simulink model "bu_abslut125_rombina_32"  (R2021b)
(part 3 of 8)

  ROM6 : hdlBasic/ROM  depth=7874  initVector=[1,0,0,0,0,1,0,1,1,1,1,1,1,0,0,1,1,0,0,1,1,1,0,0,1,1,1,0,0,0,0,1,1,0,0,0,0,0,1,1,0,0,0,1,1,0,1,1,0,0,0,1,1,1,0,1,1,0,0,0,1,1,1,0,0,1,1,1,0,0,1,1,1,0,0,1,1,1,1,0,0,1,1,1,0,0,1,1,1,0,0,0,0,1,1,1,0,0,0,1,1,0,0,0,1,0,0,1,1,0,0,0,1,1,0,0,0,1,1,1,0,1,1,0,0,0,1,1,0,0,0,1,1,1,0,0,1,1,1,0,0,1,1,1,0,0,1,1,1,0,0,1,1,1,1,0,0,1,1,1,0,0,1,1,1,0,0,1,1,1,0,1,0,0,1,1,1,0,0,1,1,1,0,0,1,1,1,0,0,0,0,0,0,1,1,0,0,0,1,1,0,0,0,1,1,0,0,0,1,1,0,0,1,1,0,0,0,1,1,0,0,0,1,1,0,0,0,1,1,1,0,0,1,1,1,0,0,1,1,0,0,0,1,1,0,0,0,1,1,1,0,0,1,0,1,1,0,0,1,1,1,0,0,1,1,1,0,0,1,1,1,0,0,1,1,1,1,1,0,0,0,1,1,0,0,1,1,1,0,0,1,1,1,0,0,1,1,1,0,0,1,1,0,0,1,1,0,0,0,1,1,0,0,0,1,1,0,0,0,1,1,0,0,0,1,1,0,0,1,1,1,0,0,1,1,0,0,0,1,1,0,0,0,1,1,0,0,0,1,1,1,1,0,0,1,1,0,0,1,1,1,0,0,1,1,0,0,0,1,1,0,0,0,1,1,1,0,0,0,0,1,1,0,0,0,1,1,0,0,1,1,1,0,0,1,1,1,0,0,1,1,1,0,0,1,1,0,0,1,1,0,0,1,1,0,0,0,1,1,0,0,1,1,1,0,0,1,1,1,0,0,1,1,1,0,0,1,1,0,0,1,1,1,0,0,1,1,0,0,0,1,1,0,0,1,1,1,0,0,1,1,1,0,0,0,0,1,1,0,0,1,1,0,0,1,1,1,0,0,1,1,0,0,0,1,1,0,0,0,1,1,0,0,0,1,1,1,1,0,0,1,1,1,0,0,1,1,0,0,1,1,1,0,0,1,1,0,0,0,1,1,0,0,0,1,1,0,0,1,1,0,0,1,1,0,0,1,1,0,0,0,1,1,0,0,1,1,1,0,0,1,1,0,0,0,1,1,1,0,0,1,1,0,0,1,1,1,0,0,1,1,0,0,1,1,0,0,0,1,1,0,0,1,1,1,0,0,1,1,1,0,0,1,1,1,1,0,0,1,1,0,0,1,1,0,0,0,1,1,0,0,1,1,0,0,0,1,1,0,0,1,1,1,0,0,1,1,1,0,0,0,0,1,1,1,0,0,1,1,0,0,1,1,0,0,1,1,1,0,0,1,1,0,0,0,1,1,0,0,0,1,1,0,0,0,1,0,0,1,1,0,0,1,1,0,0,0,1,1,0,0,1,1,0,0,1,1,1,0,0,1,1,0,0,0,1,1,0,0,0,1,1,0,0,0,1,1,0,0,1,1,0,0,1,1,0,0,1,1,1,0,0,1,1,0,0,1,1,1,0,0,1,1,0,0,0,1,1,0,0,0,0,1,1,0,0,1,1,0,0,0,1,1,0,0,1,1,0,0,1,1,0,0,0,1,1,0,0,1,1,1,0,0,1,1,1,0,0,1,1,0,1,1,0,0,1,1,0,0,1,1,0,0,1,1,1,0,0,1,1,0,0,1,1,0,0,0,1,1,0,0,1,1,1,0,0,1,1,1,0,1,1,0,0,0,1,1,0,0,1,1,0,0,1,1,0,0,1,1,0,0,0,1,1,0,0,1,1,0,0,0,1,1,0,0,1,1,1,0,0,0,1,1,0,0,1,1,0,0,1,1,0,0,1,1,1,0,0,1,1,0,0,1,1,0,0,1,1,1,0,0,1,1,0,0,0,1,1,0,0,0,1,1,1,1,0,0,1,1,0,0,1,1,0,0,1,1,0,0,1,1,0,0,0,1,1,0,0,1,1,0,0,1,1,1,0,0,1,1,0,0,0,1,1,0,0,1,0,0,1,1,1,0,0,1,1,0,0,1,1,0,0,1,1,0,0,1,1,0,0,1,1,1,0,0,1,1,0,0,1,1,1,0,0,1,1,1,0,0,1,1,0,0,1,1,0,0,1,1,0,0,1,1,0,0,1,1,1,0,0,1,1,0,0,1,1,0,0,1,1,0,0,0,1,1,0,0,1,1,1,0,0,1,1,1,1,0,0,1,1,0,0,1,1,0,0,1,1,0,0,1,1,0,0,1,1,0,0,1,1,1,0,0,1,1,0,0,1,1,0,0,0,1,1,0,0,1,1,1,0,0,1,0,0,1,1,0,0,1,1,0,0,1,1,0,0,1,1,0,0,1,1,0,0,1,1,0,0,1,1,0,0,0,1,1,0,0,1,1,0,0,0,1,1,0,0,0,1,0,0,1,1,0,0,1,1,0,0,1,1,0,0,1,1,0,0,1,1,1,0,0,1,1,0,0,1,1,0,0,1,1,0,0,1,1,1,0,0,1,1,0,0,0,1,1,0,0,0,1,1,0,0,1,1,0,0,1,1,0,0,1,1,0,0,1,1,0,0,1,1,0,0,1,1,0,0,0,1,1,0,0,1,1,0,0,1,1,1,0,0,1,1,0,0,0,0,0,1,1,0,0,1,1,0,0,1,1,0,0,1,1,0,0,1,1,0,0,1,1,0,0,1,1,0,0,1,1,0,0,1,1,1,0,0,1,1,0,0,1,1,1,0,0,1,1,0,0,1,1,0,0,1,1,0,0,1,1,0,0,1,1,0,0,1,1,0,0,1,1,0,0,1,1,0,0,1,1,0,0,1,1,0,0,1,1,0,0,0,1,1,0,0,1,1,1,0,0,1,1,0,0,1,1,0,0,1,1,0,0,1,1,0,0,1,1,0,0,1,1,0,0,1,1,0,0,1,1,0,0,0,1,1,0,0,1,1,0,0,1,1,0,0,0,1,1,0,0,0,0,1,1,0,0,1,1,0,0,1,1,0,0,1,1,0,0,1,1,0,0,1,1,0,0,1,1,0,0,1,1,0,0,1,1,0,0,1,1,0,0,0,1,1,0,0,1,1,0,0,0,1,1,0,1,1,0,0,1,1,0,0,1,1,0,0,1,1,0,0,1,1,0,0,1,1,0,0,1,1,0,0,1,1,0,0,1,1,0,0,1,1,0,0,1,1,0,0,1,1,1,0,0,1,1,0,0,0,1,1,0,0,1,1,0,0,1,1,0,0,1,1,0,0,1,1,0,0,1,1,0,0,1,1,0,0,1,1,0,0,1,1,0,0,1,1,0,0,1,1,0,0,1,1,0,0,1,1,1,0,0,1,0,1,1,0,0,1,1,0,0,1,1,0,0,1,1,0,0,1,0,0,1,1,0,0,1,1,0,0,1,1,0,0,1,1,0,0,1,1,0,0,1,1,0,0,1,1,1,0,0,1,1,0,0,1,1,1,0,1,1,0,0,1,1,0,0,1,1,0,1,1,0,0,1,1,0,0,1,1,0,0,1,1,0,0,1,1,0,0,1,1,0,0,1,1,0,0,1,1,0,0,1,1,0,0,1,1,0,0,0,1,1,0,0,0,1,1,0,0,1,1,0,1,1,0,0,1,1,0,0,1,1,0,0,1,1,0,0,1,1,0,0,1,1,0,0,1,1,0,0,1,1,0,0,1,1,0,0,1,1,0,0,1,1,0,0,1,1,0,0,0,1,0,1,1,0,0,1,0,0,1,1,0,0,1,1,0,0,1,1,0,0,1,1,0,0,1,1,0,0,1,1,0,0,1,1,0,0,1,1,0,0,1,1,0,0,1,1,0,0,1,1,0,0,1,1,0,0,1,1,0,0,1,1,0,1,1,0,0,1,1,0,0,1,1,0,0,1,1,0,0,1,1,0,0,1,1,0,0,1,1,0,0,1,1,0,0,1,0,0,1,1,0,0,1,1,0,0,1,1,0,0,1,1,0,0,1,1,1,0,0,0,1,0,0,1,1,0,0,1,1,0,0,1,1,0,0,1,1,0,0,1,1,0,0,1,1,0,0,1,1,0,0,1,1,0,1,1,0,0,1,1,0,0,1,1,0,0,1,1,0,0,1,1,0,0,1,1,0,0,1,1,0,1,0,0,1,1,0,0,1,1,0,0,1,1,0,0,1,1,0,0,1,1,0,0,1,1,0,0,1,1,0,0,1,0,0,1,1,0,0,1,1,0,0,1,1,0,0,1,1,0,0,1,1,0,0,1,1,0,0,1,1,0,0,1,0,0,1,1,0,0,1,1,0,0,1,1,0,0,1,1,0,0,1,1,0,0,1,1,0,0,1,1,0,0,1,0,0,1,1,0,0,1,1,0,0,1,1,0 ...(+11750 chars)]  distributed_mem=Block RAM  rst=off  init_reg=0  en=off  latency=1  gui_display_data_type=Boolean  arith_type=Boolean  n_bits=2  bin_pt=0  preci_type=Double  exp_width=8  frac_width=24  optimize=Area  use_rpm=on  simulation_type=fast_sim  XmcBlockStatus=1  maskContainerNames=tabcontainer1  block_type=sprom  block_config=sysgen:SPROM_config
  ROM7 : hdlBasic/ROM  depth=7874  initVector=[0,1,1,1,0,1,0,1,0,0,1,0,0,1,0,0,0,1,0,1,1,0,1,0,1,1,0,1,1,0,0,1,0,1,1,0,0,0,1,0,1,1,0,1,0,0,1,0,1,1,0,1,0,0,1,1,0,1,1,0,1,0,0,1,0,1,0,0,1,0,1,0,0,1,0,1,1,0,0,1,0,1,1,0,1,0,1,1,0,1,0,1,0,1,1,0,1,0,0,1,0,1,1,0,1,0,0,1,0,1,0,0,1,0,1,1,0,1,0,0,0,1,0,1,1,0,1,0,1,1,0,1,0,0,1,0,1,0,0,1,0,1,0,0,1,0,1,0,0,1,0,1,1,1,0,1,0,1,0,0,1,0,1,0,0,1,0,1,1,0,1,0,1,0,1,1,0,1,0,1,1,0,1,0,1,1,0,1,0,0,1,1,0,1,0,1,0,0,1,0,1,0,0,1,0,1,0,0,1,0,1,0,1,0,1,1,0,1,0,1,0,0,1,0,1,1,0,1,0,0,1,0,1,1,0,1,0,1,0,1,1,0,1,0,1,1,0,1,0,0,1,0,1,0,1,0,1,0,1,1,0,1,0,1,0,0,1,0,1,0,0,1,0,1,1,0,1,0,1,1,0,1,0,1,0,1,1,0,1,0,1,1,0,1,0,1,1,0,1,0,1,0,1,0,1,0,1,1,0,1,0,1,0,0,1,0,1,0,0,1,0,1,0,0,1,0,1,0,1,1,0,1,0,1,0,1,1,0,1,0,1,0,0,1,0,1,1,0,1,0,0,0,1,0,1,0,1,0,1,0,0,1,0,1,0,1,1,0,1,0,1,1,0,1,0,0,1,0,1,0,1,0,1,1,0,1,0,1,0,1,1,0,1,0,1,0,0,1,0,1,0,0,1,0,1,1,0,0,1,0,1,0,1,0,1,0,0,1,0,1,0,1,1,0,1,0,1,0,0,1,0,1,1,0,1,0,1,0,1,0,1,1,0,1,0,1,0,1,0,0,1,0,1,0,1,1,0,1,0,1,1,0,1,0,0,0,1,0,1,0,1,0,1,0,1,1,0,1,0,1,0,1,0,0,1,0,1,0,0,1,0,1,0,0,1,0,1,0,1,0,1,0,0,1,0,1,0,1,0,1,0,0,1,0,1,0,1,1,0,1,0,1,1,0,1,0,1,1,1,0,1,0,1,0,1,0,1,0,1,1,0,1,0,1,0,1,0,0,1,0,1,0,1,1,0,1,0,0,1,0,1,0,1,0,1,0,0,1,0,1,0,1,0,1,0,1,1,0,1,0,1,0,1,1,0,1,0,1,0,0,1,0,1,1,0,0,1,0,1,0,1,0,1,0,1,0,0,1,0,1,0,1,0,1,0,0,1,0,1,0,1,1,0,1,0,1,1,0,1,0,1,0,1,0,0,1,0,1,0,1,0,1,0,1,0,1,1,0,1,0,1,0,1,0,0,1,0,1,0,0,1,0,1,0,0,1,1,0,1,0,1,0,1,0,1,0,0,1,0,1,0,1,0,1,0,1,0,0,1,0,1,0,1,1,0,1,0,1,0,0,1,0,1,1,0,1,0,1,0,1,0,1,0,1,0,1,0,1,0,0,1,0,1,0,1,0,1,0,0,1,0,1,0,1,1,0,1,0,1,1,0,0,1,0,1,0,1,0,1,0,0,1,0,1,0,1,0,1,0,1,0,1,1,0,1,0,1,0,1,0,0,1,0,1,0,0,1,0,1,1,0,1,0,1,0,1,0,1,0,1,0,1,0,1,0,0,1,0,1,0,1,0,1,0,1,0,0,1,0,1,0,1,1,0,1,0,1,1,0,1,1,0,1,0,0,1,0,1,0,1,0,1,0,1,0,1,0,1,0,1,0,0,1,0,1,0,1,0,1,0,0,1,0,1,0,1,1,0,1,0,0,1,0,1,0,1,0,1,0,1,0,1,0,1,1,0,1,0,1,0,1,0,1,0,1,0,1,1,0,1,0,1,0,1,0,0,1,0,1,0,0,1,0,1,0,1,0,1,0,1,0,1,0,1,0,1,0,1,0,1,0,1,0,0,1,0,1,0,1,0,1,0,1,0,0,1,0,1,0,1,1,0,1,0,1,1,0,1,0,1,1,0,1,0,1,0,1,0,1,0,1,0,1,0,1,0,1,0,1,0,1,0,0,1,0,1,0,1,0,1,0,0,1,0,1,0,0,1,0,1,0,1,0,1,0,1,0,1,0,1,0,1,0,1,0,1,0,0,1,0,1,0,1,0,1,0,1,0,1,0,1,1,0,1,0,1,0,1,0,0,1,0,1,1,0,0,1,0,1,0,1,0,1,0,1,0,1,0,1,0,1,0,1,0,1,0,1,0,1,0,0,1,0,1,0,1,0,1,0,1,0,0,1,0,1,0,1,1,0,1,0,0,1,0,1,0,1,0,1,0,1,0,1,0,1,0,1,0,1,0,1,0,1,0,1,0,1,0,1,0,1,0,0,1,0,1,0,1,0,1,0,0,1,0,1,0,0,1,1,0,1,0,1,0,1,0,1,0,1,0,1,0,1,0,1,0,1,1,0,1,0,1,0,1,0,1,0,1,0,1,0,1,0,1,0,0,1,0,1,0,1,0,0,1,0,1,1,0,1,0,1,0,1,0,1,0,1,0,1,0,1,0,1,0,1,0,1,0,1,0,1,0,1,0,1,1,0,1,0,1,0,1,0,1,0,1,0,0,1,0,1,0,1,1,0,1,0,1,0,1,0,1,0,1,0,1,0,1,0,1,0,1,0,1,0,1,0,1,0,1,0,1,0,1,0,1,0,1,0,1,0,0,1,0,1,0,1,0,1,0,0,1,0,1,0,1,0,1,0,1,0,1,0,1,0,1,0,1,0,1,0,1,0,1,0,1,0,1,0,1,0,1,0,1,0,1,0,1,0,1,0,1,0,1,0,1,0,0,1,0,1,0,1,1,0,1,0,1,0,1,0,1,0,1,0,1,0,1,0,1,0,1,0,1,0,1,0,1,0,1,0,1,0,1,0,1,0,1,0,0,1,0,1,0,1,0,1,0,1,0,1,0,0,1,0,1,0,0,0,1,0,1,0,1,0,1,0,1,0,1,0,1,0,1,0,1,0,1,0,1,0,1,0,1,0,1,0,1,0,1,0,1,0,1,0,1,0,1,0,0,1,0,1,0,1,0,1,0,0,1,0,0,1,0,1,0,1,0,1,0,1,0,1,0,1,0,1,0,1,0,1,0,1,0,1,0,1,0,1,0,1,0,1,0,1,0,1,0,1,0,1,0,1,0,1,0,1,0,0,1,0,1,0,1,1,0,1,0,1,0,1,0,1,0,1,0,1,0,1,0,1,0,1,0,1,0,1,0,1,0,1,0,1,0,1,0,1,0,1,0,1,0,1,0,1,0,1,0,1,0,1,0,1,0,1,0,0,1,0,1,0,1,0,1,0,1,0,1,0,1,0,1,0,1,0,1,0,1,1,0,1,0,1,0,1,0,1,0,1,0,1,0,1,0,1,0,1,0,1,0,1,0,1,0,1,0,0,1,0,1,0,1,0,1,0,0,0,1,0,1,0,1,0,1,0,1,0,1,1,0,1,0,1,0,1,0,1,0,1,0,1,0,1,0,1,0,1,0,1,0,1,0,1,0,1,0,1,0,1,0,1,0,1,0,1,0,1,0,0,1,0,1,0,0,1,0,1,0,1,0,1,1,0,1,0,1,0,1,0,1,0,1,0,1,0,1,0,1,0,1,0,1,0,1,0,1,0,1,0,1,0,1,0,1,0,1,0,1,0,1,0,1,0,1,0,1,0,1,0,0,1,0,1,0,1,0,0,1,0,1,0,1,0,1,0,1,0,1,0,1,0,1,0,1,0,1,0,1,0,1,0,1,0,1,0,1,0,1,0,1,0,1,0,1,0,1,0,1,0,1,0,1,0,1,0,1,0,1,0,1,0,1,0,0,1,0,1,0,1,0,1,0,1,0,1,0,1,0,1,0,1,0,1,0,1,0,1,0,1,0,1,0,1,0,1,0,1,1,0,1,0,1,0,1,0,1,0,1,0,1,0,1,0,1,0,1,0,0,1,0,0,1,1,0,1,0,1,0,1,0,1,0,1,0,1,0,1,0,1,0,1,0,1,0,1,0,1,0,1,0,1,0,1,0,0,1,0,1,0,1,0,1,0,1,0,1,0,1,0,1,0,1,0,1,0,1,0,1,0,1,0,0,0,1,0,1,0,1,0,1,0,1,0,1,0,1,0,1,0,1,0,1,0,1,0,1,0,1,0,1,0,1,0,0,1,0,1,0,1,0,1,0,1,0,1,0,1,0,1,0,1,0,1,0,1,0,1,0,1,0,1,0,1,0,0,1,0,1,0,1,0,1,0,1,0,1,0,1,0,1,0,1,0,1,0,1,0,1,0,1,0,1,0,1,0,0,1,0,1,0,1,0,1,0,1,0,1,0,1 ...(+11750 chars)]  distributed_mem=Block RAM  rst=off  init_reg=0  en=off  latency=1  gui_display_data_type=Boolean  arith_type=Boolean  n_bits=2  bin_pt=0  preci_type=Double  exp_width=8  frac_width=24  optimize=Area  use_rpm=on  simulation_type=fast_sim  XmcBlockStatus=1  maskContainerNames=tabcontainer1  block_type=sprom  block_config=sysgen:SPROM_config
  ROM8 : hdlBasic/ROM  depth=7874  initVector=[1,1,0,0,0,1,0,1,1,0,1,1,0,0,1,1,0,0,1,1,0,0,0,1,1,0,0,1,1,1,0,0,1,1,0,0,1,0,0,1,1,0,0,1,1,0,0,1,1,0,0,1,1,0,0,1,1,1,0,0,1,1,0,0,1,1,1,0,0,1,1,1,0,0,1,1,0,0,0,0,1,1,0,0,0,1,1,0,0,1,1,1,1,1,0,0,1,1,0,0,1,1,0,0,1,1,0,0,1,1,1,0,0,1,1,0,0,1,1,0,0,0,1,1,0,0,0,1,1,0,0,1,1,0,0,1,1,1,0,0,0,1,1,0,0,0,1,1,0,0,1,1,0,0,0,0,1,1,1,0,0,1,1,1,0,0,1,1,0,0,1,0,1,1,1,0,0,1,1,1,0,0,1,1,1,0,0,1,1,0,1,0,0,0,1,1,1,0,0,0,1,1,0,0,1,1,1,0,1,1,0,0,1,1,1,0,0,0,1,1,1,0,0,1,1,0,0,1,1,0,0,1,1,0,0,0,0,1,1,1,0,0,1,1,1,0,0,1,1,0,0,1,1,0,0,0,1,1,1,0,0,0,1,1,1,0,0,0,1,1,0,0,1,1,0,0,1,1,1,0,0,0,0,1,1,1,0,0,0,1,1,0,0,0,1,1,0,0,1,1,0,0,0,0,1,1,1,0,0,0,0,1,1,0,0,0,1,1,0,0,0,1,1,0,0,1,1,1,1,0,0,0,0,1,1,1,0,0,0,1,1,1,0,0,1,1,0,0,0,1,0,0,0,0,0,0,1,1,1,1,0,0,0,1,1,1,0,0,0,1,1,0,0,1,1,0,0,1,0,1,1,1,1,0,0,0,0,1,1,1,0,0,0,0,1,1,0,0,0,1,1,0,0,1,1,0,1,0,0,0,0,1,1,1,1,1,0,0,0,1,1,1,0,0,0,1,1,1,0,0,1,1,0,0,1,1,1,1,1,1,1,0,0,0,0,1,1,1,1,0,0,0,1,1,1,0,0,1,1,1,0,0,1,1,0,0,0,0,0,0,0,1,1,1,1,0,0,0,0,1,1,1,1,0,0,1,1,1,0,0,0,1,1,0,0,1,1,1,1,1,1,1,0,0,0,0,0,1,1,1,1,0,0,0,1,1,1,0,0,0,1,1,0,0,0,1,1,0,0,0,0,0,0,0,1,1,1,1,1,0,0,0,0,1,1,1,1,0,0,0,1,1,1,0,0,1,1,0,0,1,1,1,1,1,1,1,0,0,0,0,0,0,1,1,1,1,0,0,0,0,1,1,1,0,0,0,1,1,1,0,0,1,1,0,0,0,0,0,0,0,1,1,1,1,1,1,0,0,0,0,0,1,1,1,1,0,0,0,1,1,1,0,0,0,1,1,0,0,1,1,1,1,1,1,0,0,0,0,0,0,0,1,1,1,1,1,0,0,0,0,1,1,1,1,0,0,0,1,1,0,0,0,1,1,0,0,0,0,1,1,1,1,1,1,1,1,0,0,0,0,0,0,1,1,1,1,1,0,0,0,1,1,1,0,0,0,1,1,1,0,0,1,1,0,0,0,0,0,0,0,0,0,0,1,1,1,1,1,1,0,0,0,0,0,1,1,1,1,0,0,0,1,1,1,0,0,1,1,1,0,0,1,1,1,1,1,1,1,1,1,0,0,0,0,0,0,0,1,1,1,1,1,0,0,0,0,1,1,1,1,0,0,0,1,1,0,0,1,1,0,0,0,0,0,0,0,0,1,1,1,1,1,1,1,1,0,0,0,0,0,0,1,1,1,1,1,0,0,0,1,1,1,0,0,0,1,1,0,0,1,1,1,1,1,0,0,0,0,0,0,0,0,0,0,1,1,1,1,1,1,1,0,0,0,0,0,1,1,1,1,0,0,0,1,1,1,0,0,1,1,0,1,1,1,1,1,1,1,1,1,1,1,1,1,0,0,0,0,0,0,0,0,1,1,1,1,1,0,0,0,0,1,1,1,1,0,0,0,1,1,0,0,1,0,0,0,0,0,0,0,0,0,0,1,1,1,1,1,1,1,1,1,1,0,0,0,0,0,0,1,1,1,1,1,0,0,0,1,1,1,0,0,0,1,1,0,1,1,1,1,0,0,0,0,0,0,0,0,0,0,0,0,0,0,0,1,1,1,1,1,1,1,0,0,0,0,0,1,1,1,1,0,0,0,1,1,0,0,0,1,1,1,1,1,1,1,1,1,1,1,1,1,1,1,1,1,1,0,0,0,0,0,0,0,0,0,1,1,1,1,1,0,0,0,0,0,1,1,1,0,0,1,1,0,0,0,0,0,0,0,0,0,0,0,0,0,0,1,1,1,1,1,1,1,1,1,1,1,1,1,0,0,0,0,0,0,0,1,1,1,1,0,0,0,1,1,1,0,0,1,1,0,0,0,0,0,0,0,0,0,0,0,0,0,0,0,0,0,0,0,0,0,0,0,1,1,1,1,1,1,1,1,0,0,0,0,0,1,1,1,1,0,0,0,1,1,0,0,1,1,1,1,1,1,1,1,1,1,1,1,1,1,1,1,1,1,1,0,0,0,0,0,0,0,0,0,0,0,0,1,1,1,1,1,1,0,0,0,0,1,1,1,0,0,1,1,1,1,1,1,1,1,1,1,1,1,1,1,1,1,1,1,1,1,1,1,1,1,1,1,1,1,1,1,1,0,0,0,0,0,0,0,0,1,1,1,1,0,0,0,1,1,1,0,0,0,0,0,0,0,0,0,0,0,0,0,0,0,0,0,0,0,0,0,0,0,0,0,0,0,0,1,1,1,1,1,1,1,1,1,1,0,0,0,0,0,0,1,1,1,0,0,0,1,1,0,0,0,0,0,0,0,0,0,0,0,0,0,0,0,0,0,0,0,0,0,0,0,0,0,0,0,0,0,0,0,0,0,0,0,0,1,1,1,1,1,1,0,0,0,0,1,1,0,0,1,1,1,1,1,1,1,1,1,1,1,1,1,1,1,1,1,1,1,1,1,1,1,1,1,1,1,1,1,1,1,1,1,1,0,0,0,0,0,0,0,0,0,1,1,1,1,0,0,0,1,1,0,1,1,1,1,1,1,1,1,1,1,1,1,1,1,1,1,1,1,1,1,1,1,1,1,1,1,1,1,1,1,1,1,1,1,1,1,1,1,1,1,1,0,0,0,0,0,0,1,1,1,0,0,1,1,1,1,1,1,1,1,1,1,0,0,0,0,0,0,0,0,0,0,0,0,0,0,0,0,0,0,0,0,0,0,0,0,0,0,0,0,0,0,0,1,1,1,1,1,1,1,0,0,0,0,1,1,0,1,1,0,0,0,0,0,0,0,0,0,0,0,0,0,0,0,0,0,0,0,0,0,0,0,0,0,0,0,0,0,0,0,0,0,0,0,0,0,0,0,0,0,0,0,0,0,1,1,1,1,0,0,0,1,0,0,0,0,0,0,0,0,0,0,0,0,0,0,0,0,0,0,1,1,1,1,1,1,1,1,1,1,1,1,1,1,1,1,1,1,1,1,1,1,1,1,1,1,1,1,0,0,0,0,0,0,1,1,1,0,0,0,0,0,0,0,0,0,0,0,0,0,1,1,1,1,1,1,1,1,1,1,1,1,1,1,1,1,1,1,1,1,1,1,1,1,1,1,1,1,1,1,1,1,1,1,1,1,1,1,1,1,0,0,0,1,1,0,0,0,0,0,0,0,0,1,1,1,1,1,1,1,1,1,1,1,1,1,1,1,1,1,1,1,0,0,0,0,0,0,0,0,0,0,0,0,0,0,0,0,0,0,0,0,0,0,0,0,0,1,1,1,1,0,0,0,0,0,0,0,1,1,1,1,1,1,1,1,1,1,1,1,1,1,1,1,1,0,0,0,0,0,0,0,0,0,0,0,0,0,0,0,0,0,0,0,0,0,0,0,0,0,0,0,0,0,0,0,0,0,0,0,1,1,0,0,0,1,1,1,1,1,1,1,1,1,1,1,1,1,1,1,1,0,0,0,0,0,0,0,0,0,0,0,0,0,0,0,0,0,0,1,1,1,1,1,1,1,1,1,1,1,1,1,1,1,1,1,1,1,1,0,0,0,0,0,1,1,1,1,1,1,1,1,1,1,1,1,1,1,1,0,0,0,0,0,0,0,0,0,0,0,0,0,0,0,0,0,1,1,1,1,1,1,1,1,1,1,1,1,1,1,1,1,1,1,1,1,1,1,1,1,1,1,1,0,1,1,1,1,1,1,1,1,1,1,1,1,1,1,1,0,0,0,0,0,0,0,0,0,0,0,0,0,0,0,0,1,1,1,1,1,1,1,1,1,1,1,1,1,1,1,1,0,0,0,0,0,0,0,0,0,0,0,0,0,0,0,1,1,1,1,1,1,1,1,1,1,1,1,1,1,1,0,0,0,0,0,0,0,0,0,0,0,0,0,0,0,0,1,1,1,1,1,1,1,1,1,1,1,1,1,1 ...(+11750 chars)]  distributed_mem=Block RAM  rst=off  init_reg=0  en=off  latency=1  gui_display_data_type=Boolean  arith_type=Boolean  n_bits=2  bin_pt=0  preci_type=Double  exp_width=8  frac_width=24  optimize=Area  use_rpm=on  simulation_type=fast_sim  XmcBlockStatus=1  maskContainerNames=tabcontainer1  block_type=sprom  block_config=sysgen:SPROM_config
  ROM9 : hdlBasic/ROM  depth=7874  initVector=[0,1,0,0,1,0,1,0,1,0,0,1,0,1,0,1,0,1,0,1,0,0,1,0,1,0,1,1,0,1,0,1,0,1,0,1,1,0,1,0,1,0,1,0,1,0,1,0,1,0,1,0,1,0,1,0,0,1,0,1,0,1,0,1,0,1,1,0,1,0,0,1,0,1,0,1,0,1,0,1,0,1,0,1,1,0,1,0,1,0,1,0,1,1,0,1,0,1,0,1,0,1,0,1,0,1,0,1,0,0,1,0,1,0,1,0,1,0,1,0,1,1,0,1,0,1,1,0,1,0,1,0,1,0,1,0,0,1,0,0,1,0,1,0,0,1,0,1,0,1,0,1,0,0,0,1,0,1,1,0,1,0,1,1,0,1,0,1,0,1,0,1,0,1,1,0,1,0,0,1,0,1,0,1,1,0,1,0,1,0,1,0,0,1,0,0,1,0,1,1,0,1,0,1,0,1,1,0,0,1,1,1,0,1,1,0,1,1,0,1,1,0,1,0,1,0,1,0,1,0,1,0,1,0,0,1,1,0,1,1,0,1,0,0,1,0,1,0,1,0,1,0,1,0,1,1,0,0,1,0,0,1,0,0,1,0,1,1,0,1,0,1,0,1,0,1,0,0,1,0,0,1,1,0,1,1,0,1,1,0,1,0,1,1,0,1,0,1,0,1,0,0,1,1,0,0,1,0,0,1,1,0,1,0,0,1,0,1,0,0,1,0,1,0,1,0,0,1,1,0,0,1,1,0,0,1,0,0,1,0,0,1,0,1,0,1,0,0,1,0,0,0,0,0,1,1,0,0,1,1,0,1,1,0,1,1,0,1,1,0,1,0,1,0,1,0,1,0,1,0,0,1,1,0,0,1,1,0,0,1,0,0,1,1,0,1,0,0,1,0,1,0,1,0,1,0,1,0,0,1,1,0,0,0,1,1,0,1,1,0,0,1,0,0,1,0,1,1,0,1,0,1,0,1,0,0,0,0,1,1,1,0,0,1,1,0,0,1,1,0,1,1,0,1,1,0,1,0,0,1,0,1,0,1,0,0,0,0,1,1,1,0,0,1,1,0,0,1,1,0,0,1,1,0,1,0,0,1,0,1,1,0,1,0,1,0,0,0,0,1,1,1,0,0,1,1,1,0,0,1,1,0,1,1,0,0,1,0,0,1,0,1,0,1,1,0,1,1,0,0,0,1,1,1,0,0,1,1,1,0,0,1,1,0,0,1,1,0,1,1,0,1,1,0,1,0,1,0,1,0,1,0,0,1,1,1,0,0,0,1,1,1,0,0,1,1,0,0,1,1,0,0,1,0,0,1,0,0,1,0,1,0,1,0,1,0,1,1,1,1,0,0,0,1,1,1,0,0,1,1,1,0,0,1,1,0,1,1,0,0,1,0,1,1,0,1,0,1,0,1,1,1,1,1,0,0,0,0,1,1,1,0,0,1,1,1,0,0,1,1,0,0,1,1,0,1,1,0,1,0,0,1,0,1,0,1,1,1,0,0,0,0,0,1,1,1,0,0,0,1,1,1,0,0,1,1,1,0,0,1,0,0,1,0,0,1,0,1,1,0,1,0,1,0,0,0,0,0,0,1,1,1,1,0,0,0,1,1,1,0,0,0,1,1,0,0,1,1,0,0,1,0,0,1,0,1,0,0,1,0,1,0,0,0,0,1,1,1,1,1,0,0,0,1,1,1,1,0,0,0,1,1,0,0,1,1,0,0,1,1,0,1,1,0,1,0,1,0,1,0,1,1,1,1,1,1,1,0,0,0,0,1,1,1,1,0,0,0,1,1,1,0,0,0,1,1,0,0,1,0,0,1,0,0,1,0,1,0,1,0,1,1,1,1,0,0,0,0,0,0,1,1,1,1,0,0,0,0,1,1,1,0,0,0,1,1,0,0,1,1,0,0,1,0,1,1,0,1,0,1,0,0,0,0,0,0,0,0,1,1,1,1,1,1,0,0,0,0,1,1,1,1,0,0,0,1,1,0,0,1,1,0,0,1,1,0,1,1,0,1,0,1,0,0,1,1,1,1,1,1,1,1,1,0,0,0,0,0,0,1,1,1,1,0,0,0,0,1,1,0,0,0,1,1,0,0,1,0,0,1,0,0,1,0,1,0,1,1,1,1,0,0,0,0,0,0,0,0,0,1,1,1,1,1,1,0,0,0,0,1,1,1,0,0,0,1,1,0,0,1,1,0,0,1,0,1,0,0,1,0,0,0,0,0,0,0,0,0,1,1,1,1,1,1,1,1,1,0,0,0,0,0,1,1,1,1,0,0,0,1,1,0,0,0,1,1,0,1,1,0,1,0,1,0,1,1,1,1,1,1,1,1,1,1,1,1,1,0,0,0,0,0,0,0,0,1,1,1,1,1,0,0,0,0,1,1,1,0,0,1,1,0,0,1,0,0,1,0,1,0,1,0,0,0,0,0,0,0,0,0,0,0,0,0,0,0,1,1,1,1,1,1,1,1,0,0,0,0,0,1,1,1,0,0,0,1,1,0,0,1,1,0,1,1,0,1,0,1,1,1,1,1,1,1,1,1,1,1,1,1,1,1,1,1,1,1,1,0,0,0,0,0,0,0,1,1,1,1,1,0,0,0,1,1,1,0,0,1,1,0,1,1,0,1,0,1,0,0,0,0,0,0,0,0,0,0,0,0,0,0,0,0,0,0,0,0,0,0,0,1,1,1,1,1,1,0,0,0,0,0,1,1,1,0,0,1,1,0,0,1,0,0,1,0,1,1,1,1,1,1,1,1,1,1,1,1,1,1,1,1,1,1,1,1,1,1,1,1,1,1,1,0,0,0,0,0,0,1,1,1,1,0,0,0,1,1,1,0,1,1,0,1,1,0,1,0,0,0,0,0,0,0,0,0,0,0,0,0,0,0,0,0,0,0,0,0,0,0,0,0,0,0,0,0,0,1,1,1,1,1,1,0,0,0,1,1,1,0,0,1,1,0,1,0,1,0,1,1,1,1,1,1,1,1,1,1,1,1,1,1,1,1,1,1,1,1,1,1,1,1,1,1,1,1,1,1,1,1,1,0,0,0,0,0,1,1,1,1,0,0,1,1,0,0,1,0,1,0,1,1,1,1,1,0,0,0,0,0,0,0,0,0,0,0,0,0,0,0,0,0,0,0,0,0,0,0,0,0,0,0,0,0,0,0,1,1,1,1,1,0,0,0,1,1,1,0,1,1,0,1,0,0,0,0,0,0,0,0,0,0,1,1,1,1,1,1,1,1,1,1,1,1,1,1,1,1,1,1,1,1,1,1,1,1,1,1,1,1,1,1,1,0,0,0,0,1,1,1,0,0,1,1,0,1,0,0,0,1,1,1,1,1,1,1,1,1,1,1,1,0,0,0,0,0,0,0,0,0,0,0,0,0,0,0,0,0,0,0,0,0,0,0,0,0,0,0,0,0,1,1,1,1,0,0,1,1,0,0,1,0,1,1,1,1,1,1,1,0,0,0,0,0,0,0,0,0,0,0,1,1,1,1,1,1,1,1,1,1,1,1,1,1,1,1,1,1,1,1,1,1,1,1,1,1,1,1,0,0,0,0,1,1,0,1,1,0,1,1,0,0,0,0,0,0,0,0,0,0,1,1,1,1,1,1,1,1,1,1,1,0,0,0,0,0,0,0,0,0,0,0,0,0,0,0,0,0,0,0,0,0,0,0,0,0,0,1,1,1,0,0,1,0,1,0,0,0,0,0,0,0,0,1,1,1,1,1,1,1,1,1,0,0,0,0,0,0,0,0,0,0,1,1,1,1,1,1,1,1,1,1,1,1,1,1,1,1,1,1,1,1,1,1,1,1,1,0,0,0,1,0,1,0,0,0,0,0,1,1,1,1,1,1,1,1,0,0,0,0,0,0,0,0,0,1,1,1,1,1,1,1,1,1,1,0,0,0,0,0,0,0,0,0,0,0,0,0,0,0,0,0,0,0,0,0,0,0,1,1,0,1,0,0,0,1,1,1,1,1,1,1,1,0,0,0,0,0,0,0,0,1,1,1,1,1,1,1,1,1,0,0,0,0,0,0,0,0,0,1,1,1,1,1,1,1,1,1,1,1,1,1,1,1,1,1,1,1,1,0,0,1,0,0,1,1,1,1,1,1,1,0,0,0,0,0,0,0,0,1,1,1,1,1,1,1,1,0,0,0,0,0,0,0,0,0,1,1,1,1,1,1,1,1,0,0,0,0,0,0,0,0,0,0,0,0,0,0,0,0,0,0,1,0,1,1,1,1,1,1,1,1,0,0,0,0,0,0,0,1,1,1,1,1,1,1,1,0,0,0,0,0,0,0,0,1,1,1,1,1,1,1,1,0,0,0,0,0,0,0,0,1,1,1,1,1,1,1,1,1,1,1,1,1,1,0,1,1,1,1,1,1,1,0,0,0,0,0,0,0,0,1,1,1,1,1,1,1,1,0,0,0,0,0,0,0,0,1,1,1,1,1,1,1,0,0,0,0,0,0,0 ...(+11750 chars)]  distributed_mem=Block RAM  rst=off  init_reg=0  en=off  latency=1  gui_display_data_type=Boolean  arith_type=Boolean  n_bits=2  bin_pt=0  preci_type=Double  exp_width=8  frac_width=24  optimize=Area  use_rpm=on  simulation_type=fast_sim  XmcBlockStatus=1  maskContainerNames=tabcontainer1  block_type=sprom  block_config=sysgen:SPROM_config
  Relational : hdlBasic/Relational  mode=a<b  op_type=Bool  en=off  latency=1  XmcBlockStatus=1  maskContainerNames=tabcontainer1  block_type=relational  block_config=sysgen:Relational_config
  Relational{1..92,95..118,120..122,124..208,210,238..239,250,253,258..262,264..273,275..284,286..295,297..302} (250 alike) : hdlBasic/Relational  mode=a>=b  op_type=Bool  en=off  latency=1  XmcBlockStatus=1  maskContainerNames=tabcontainer1  block_type=relational  block_config=sysgen:Relational_config
  Scaling : hdlBasic/Scale  scale_factor=-31  XmcBlockStatus=1  maskContainerNames=group1  block_type=scale  block_config=sysgen:Scale_config
  Slice : hdlBasic/Slice  nbits=7  boolean_output=off  mode=Lower Bit Location + Width  bit1=-1  base1=MSB of Input  bit0=0  base0=LSB of Input  XmcBlockStatus=1  maskContainerNames=group1  block_type=slice  block_config=sysgen:Slice_config
  Slice1 : hdlBasic/Slice  nbits=7  boolean_output=off  mode=Lower Bit Location + Width  bit1=-1  base1=MSB of Input  bit0=0  base0=LSB of Input  XmcBlockStatus=1  maskContainerNames=group1  block_type=slice  block_config=sysgen:Slice_config
  Slice2 : hdlBasic/Slice  nbits=21  boolean_output=off  mode=Two Bit Locations  bit1=-1  base1=MSB of Input  bit0=1  base0=LSB of Input  XmcBlockStatus=1  maskContainerNames=group1  block_type=slice  block_config=sysgen:Slice_config
  Slice3 : hdlBasic/Slice  nbits=21  boolean_output=off  mode=Two Bit Locations  bit1=-4  base1=MSB of Input  bit0=0  base0=LSB of Input  XmcBlockStatus=1  maskContainerNames=group1  block_type=slice  block_config=sysgen:Slice_config
  logi_b0 : hdlBasic/Constant  const=-1.0000000000000000000000000000000000000000000000000000000  gui_display_data_type=Fixed-point  arith_type=Signed (2's comp)  n_bits=32  bin_pt=30  preci_type=Double  exp_width=8  frac_width=24  explicit_period=on  period=1  XmcBlockStatus=1  maskContainerNames=tabcontainer1  block_type=constant  block_config=sysgen:Constant_config
  logi_b1 : hdlBasic/Constant  const=-0.9838709677419354981964261241955682635307312011718750000  gui_display_data_type=Fixed-point  arith_type=Signed (2's comp)  n_bits=32  bin_pt=30  preci_type=Double  exp_width=8  frac_width=24  explicit_period=on  period=1  XmcBlockStatus=1  maskContainerNames=tabcontainer1  block_type=constant  block_config=sysgen:Constant_config
  logi_b10 : hdlBasic/Constant  const=-0.8387096774193547599196563169243745505809783935546875000  gui_display_data_type=Fixed-point  arith_type=Signed (2's comp)  n_bits=32  bin_pt=30  preci_type=Double  exp_width=8  frac_width=24  explicit_period=on  period=1  XmcBlockStatus=1  maskContainerNames=tabcontainer1  block_type=constant  block_config=sysgen:Constant_config
  logi_b100 : hdlBasic/Constant  const=0.6129032258064516236473195931466761976480484008789062500  gui_display_data_type=Fixed-point  arith_type=Signed (2's comp)  n_bits=32  bin_pt=30  preci_type=Double  exp_width=8  frac_width=24  explicit_period=on  period=1  XmcBlockStatus=1  maskContainerNames=tabcontainer1  block_type=constant  block_config=sysgen:Constant_config
  logi_b101 : hdlBasic/Constant  const=0.6290322580645161254508934689511079341173171997070312500  gui_display_data_type=Fixed-point  arith_type=Signed (2's comp)  n_bits=32  bin_pt=30  preci_type=Double  exp_width=8  frac_width=24  explicit_period=on  period=1  XmcBlockStatus=1  maskContainerNames=tabcontainer1  block_type=constant  block_config=sysgen:Constant_config
  logi_b102 : hdlBasic/Constant  const=0.6451612903225806272544673447555396705865859985351562500  gui_display_data_type=Fixed-point  arith_type=Signed (2's comp)  n_bits=32  bin_pt=30  preci_type=Double  exp_width=8  frac_width=24  explicit_period=on  period=1  XmcBlockStatus=1  maskContainerNames=tabcontainer1  block_type=constant  block_config=sysgen:Constant_config
  logi_b103 : hdlBasic/Constant  const=0.6612903225806451290580412205599714070558547973632812500  gui_display_data_type=Fixed-point  arith_type=Signed (2's comp)  n_bits=32  bin_pt=30  preci_type=Double  exp_width=8  frac_width=24  explicit_period=on  period=1  XmcBlockStatus=1  maskContainerNames=tabcontainer1  block_type=constant  block_config=sysgen:Constant_config
  logi_b104 : hdlBasic/Constant  const=0.6774193548387096308616150963644031435251235961914062500  gui_display_data_type=Fixed-point  arith_type=Signed (2's comp)  n_bits=32  bin_pt=30  preci_type=Double  exp_width=8  frac_width=24  explicit_period=on  period=1  XmcBlockStatus=1  maskContainerNames=tabcontainer1  block_type=constant  block_config=sysgen:Constant_config
  logi_b105 : hdlBasic/Constant  const=0.6935483870967741326651889721688348799943923950195312500  gui_display_data_type=Fixed-point  arith_type=Signed (2's comp)  n_bits=32  bin_pt=30  preci_type=Double  exp_width=8  frac_width=24  explicit_period=on  period=1  XmcBlockStatus=1  maskContainerNames=tabcontainer1  block_type=constant  block_config=sysgen:Constant_config
  logi_b106 : hdlBasic/Constant  const=0.7096774193548387454910653104889206588268280029296875000  gui_display_data_type=Fixed-point  arith_type=Signed (2's comp)  n_bits=32  bin_pt=30  preci_type=Double  exp_width=8  frac_width=24  explicit_period=on  period=1  XmcBlockStatus=1  maskContainerNames=tabcontainer1  block_type=constant  block_config=sysgen:Constant_config
  logi_b107 : hdlBasic/Constant  const=0.7258064516129032472946391862933523952960968017578125000  gui_display_data_type=Fixed-point  arith_type=Signed (2's comp)  n_bits=32  bin_pt=30  preci_type=Double  exp_width=8  frac_width=24  explicit_period=on  period=1  XmcBlockStatus=1  maskContainerNames=tabcontainer1  block_type=constant  block_config=sysgen:Constant_config
  logi_b108 : hdlBasic/Constant  const=0.7419354838709677490982130620977841317653656005859375000  gui_display_data_type=Fixed-point  arith_type=Signed (2's comp)  n_bits=32  bin_pt=30  preci_type=Double  exp_width=8  frac_width=24  explicit_period=on  period=1  XmcBlockStatus=1  maskContainerNames=tabcontainer1  block_type=constant  block_config=sysgen:Constant_config
  logi_b109 : hdlBasic/Constant  const=0.7580645161290322509017869379022158682346343994140625000  gui_display_data_type=Fixed-point  arith_type=Signed (2's comp)  n_bits=32  bin_pt=30  preci_type=Double  exp_width=8  frac_width=24  explicit_period=on  period=1  XmcBlockStatus=1  maskContainerNames=tabcontainer1  block_type=constant  block_config=sysgen:Constant_config
  logi_b11 : hdlBasic/Constant  const=-0.8225806451612902581160824411199428141117095947265625000  gui_display_data_type=Fixed-point  arith_type=Signed (2's comp)  n_bits=32  bin_pt=30  preci_type=Double  exp_width=8  frac_width=24  explicit_period=on  period=1  XmcBlockStatus=1  maskContainerNames=tabcontainer1  block_type=constant  block_config=sysgen:Constant_config
  logi_b110 : hdlBasic/Constant  const=0.7741935483870967527053608137066476047039031982421875000  gui_display_data_type=Fixed-point  arith_type=Signed (2's comp)  n_bits=32  bin_pt=30  preci_type=Double  exp_width=8  frac_width=24  explicit_period=on  period=1  XmcBlockStatus=1  maskContainerNames=tabcontainer1  block_type=constant  block_config=sysgen:Constant_config
  logi_b111 : hdlBasic/Constant  const=0.7903225806451612545089346895110793411731719970703125000  gui_display_data_type=Fixed-point  arith_type=Signed (2's comp)  n_bits=32  bin_pt=30  preci_type=Double  exp_width=8  frac_width=24  explicit_period=on  period=1  XmcBlockStatus=1  maskContainerNames=tabcontainer1  block_type=constant  block_config=sysgen:Constant_config
  logi_b112 : hdlBasic/Constant  const=0.8064516129032257563125085653155110776424407958984375000  gui_display_data_type=Fixed-point  arith_type=Signed (2's comp)  n_bits=32  bin_pt=30  preci_type=Double  exp_width=8  frac_width=24  explicit_period=on  period=1  XmcBlockStatus=1  maskContainerNames=tabcontainer1  block_type=constant  block_config=sysgen:Constant_config
  logi_b113 : hdlBasic/Constant  const=0.8225806451612902581160824411199428141117095947265625000  gui_display_data_type=Fixed-point  arith_type=Signed (2's comp)  n_bits=32  bin_pt=30  preci_type=Double  exp_width=8  frac_width=24  explicit_period=on  period=1  XmcBlockStatus=1  maskContainerNames=tabcontainer1  block_type=constant  block_config=sysgen:Constant_config
  logi_b114 : hdlBasic/Constant  const=0.8387096774193547599196563169243745505809783935546875000  gui_display_data_type=Fixed-point  arith_type=Signed (2's comp)  n_bits=32  bin_pt=30  preci_type=Double  exp_width=8  frac_width=24  explicit_period=on  period=1  XmcBlockStatus=1  maskContainerNames=tabcontainer1  block_type=constant  block_config=sysgen:Constant_config
  logi_b115 : hdlBasic/Constant  const=0.8548387096774193727455326552444603294134140014648437500  gui_display_data_type=Fixed-point  arith_type=Signed (2's comp)  n_bits=32  bin_pt=30  preci_type=Double  exp_width=8  frac_width=24  explicit_period=on  period=1  XmcBlockStatus=1  maskContainerNames=tabcontainer1  block_type=constant  block_config=sysgen:Constant_config
  logi_b116 : hdlBasic/Constant  const=0.8709677419354838745491065310488920658826828002929687500  gui_display_data_type=Fixed-point  arith_type=Signed (2's comp)  n_bits=32  bin_pt=30  preci_type=Double  exp_width=8  frac_width=24  explicit_period=on  period=1  XmcBlockStatus=1  maskContainerNames=tabcontainer1  block_type=constant  block_config=sysgen:Constant_config
  logi_b117 : hdlBasic/Constant  const=0.8870967741935483763526804068533238023519515991210937500  gui_display_data_type=Fixed-point  arith_type=Signed (2's comp)  n_bits=32  bin_pt=30  preci_type=Double  exp_width=8  frac_width=24  explicit_period=on  period=1  XmcBlockStatus=1  maskContainerNames=tabcontainer1  block_type=constant  block_config=sysgen:Constant_config
  logi_b118 : hdlBasic/Constant  const=0.9032258064516128781562542826577555388212203979492187500  gui_display_data_type=Fixed-point  arith_type=Signed (2's comp)  n_bits=32  bin_pt=30  preci_type=Double  exp_width=8  frac_width=24  explicit_period=on  period=1  XmcBlockStatus=1  maskContainerNames=tabcontainer1  block_type=constant  block_config=sysgen:Constant_config
  logi_b119 : hdlBasic/Constant  const=0.9193548387096773799598281584621872752904891967773437500  gui_display_data_type=Fixed-point  arith_type=Signed (2's comp)  n_bits=32  bin_pt=30  preci_type=Double  exp_width=8  frac_width=24  explicit_period=on  period=1  XmcBlockStatus=1  maskContainerNames=tabcontainer1  block_type=constant  block_config=sysgen:Constant_config
  logi_b12 : hdlBasic/Constant  const=-0.8064516129032257563125085653155110776424407958984375000  gui_display_data_type=Fixed-point  arith_type=Signed (2's comp)  n_bits=32  bin_pt=30  preci_type=Double  exp_width=8  frac_width=24  explicit_period=on  period=1  XmcBlockStatus=1  maskContainerNames=tabcontainer1  block_type=constant  block_config=sysgen:Constant_config
  logi_b120 : hdlBasic/Constant  const=0.9354838709677418817634020342666190117597579956054687500  gui_display_data_type=Fixed-point  arith_type=Signed (2's comp)  n_bits=32  bin_pt=30  preci_type=Double  exp_width=8  frac_width=24  explicit_period=on  period=1  XmcBlockStatus=1  maskContainerNames=tabcontainer1  block_type=constant  block_config=sysgen:Constant_config
  logi_b121 : hdlBasic/Constant  const=0.9516129032258063835669759100710507482290267944335937500  gui_display_data_type=Fixed-point  arith_type=Signed (2's comp)  n_bits=32  bin_pt=30  preci_type=Double  exp_width=8  frac_width=24  explicit_period=on  period=1  XmcBlockStatus=1  maskContainerNames=tabcontainer1  block_type=constant  block_config=sysgen:Constant_config
  logi_b122 : hdlBasic/Constant  const=0.9677419354838709963928522483911365270614624023437500000  gui_display_data_type=Fixed-point  arith_type=Signed (2's comp)  n_bits=32  bin_pt=30  preci_type=Double  exp_width=8  frac_width=24  explicit_period=on  period=1  XmcBlockStatus=1  maskContainerNames=tabcontainer1  block_type=constant  block_config=sysgen:Constant_config
  logi_b123 : hdlBasic/Constant  const=0.9838709677419354981964261241955682635307312011718750000  gui_display_data_type=Fixed-point  arith_type=Signed (2's comp)  n_bits=32  bin_pt=30  preci_type=Double  exp_width=8  frac_width=24  explicit_period=on  period=1  XmcBlockStatus=1  maskContainerNames=tabcontainer1  block_type=constant  block_config=sysgen:Constant_config
  logi_b124 : hdlBasic/Constant  const=1.0000000000000000000000000000000000000000000000000000000  gui_display_data_type=Fixed-point  arith_type=Signed (2's comp)  n_bits=32  bin_pt=30  preci_type=Double  exp_width=8  frac_width=24  explicit_period=on  period=1  XmcBlockStatus=1  maskContainerNames=tabcontainer1  block_type=constant  block_config=sysgen:Constant_config
  logi_b13 : hdlBasic/Constant  const=-0.7903225806451612545089346895110793411731719970703125000  gui_display_data_type=Fixed-point  arith_type=Signed (2's comp)  n_bits=32  bin_pt=30  preci_type=Double  exp_width=8  frac_width=24  explicit_period=on  period=1  XmcBlockStatus=1  maskContainerNames=tabcontainer1  block_type=constant  block_config=sysgen:Constant_config
  logi_b14 : hdlBasic/Constant  const=-0.7741935483870967527053608137066476047039031982421875000  gui_display_data_type=Fixed-point  arith_type=Signed (2's comp)  n_bits=32  bin_pt=30  preci_type=Double  exp_width=8  frac_width=24  explicit_period=on  period=1  XmcBlockStatus=1  maskContainerNames=tabcontainer1  block_type=constant  block_config=sysgen:Constant_config
  logi_b15 : hdlBasic/Constant  const=-0.7580645161290322509017869379022158682346343994140625000  gui_display_data_type=Fixed-point  arith_type=Signed (2's comp)  n_bits=32  bin_pt=30  preci_type=Double  exp_width=8  frac_width=24  explicit_period=on  period=1  XmcBlockStatus=1  maskContainerNames=tabcontainer1  block_type=constant  block_config=sysgen:Constant_config
  logi_b16 : hdlBasic/Constant  const=-0.7419354838709677490982130620977841317653656005859375000  gui_display_data_type=Fixed-point  arith_type=Signed (2's comp)  n_bits=32  bin_pt=30  preci_type=Double  exp_width=8  frac_width=24  explicit_period=on  period=1  XmcBlockStatus=1  maskContainerNames=tabcontainer1  block_type=constant  block_config=sysgen:Constant_config
  logi_b17 : hdlBasic/Constant  const=-0.7258064516129032472946391862933523952960968017578125000  gui_display_data_type=Fixed-point  arith_type=Signed (2's comp)  n_bits=32  bin_pt=30  preci_type=Double  exp_width=8  frac_width=24  explicit_period=on  period=1  XmcBlockStatus=1  maskContainerNames=tabcontainer1  block_type=constant  block_config=sysgen:Constant_config
  logi_b18 : hdlBasic/Constant  const=-0.7096774193548387454910653104889206588268280029296875000  gui_display_data_type=Fixed-point  arith_type=Signed (2's comp)  n_bits=32  bin_pt=30  preci_type=Double  exp_width=8  frac_width=24  explicit_period=on  period=1  XmcBlockStatus=1  maskContainerNames=tabcontainer1  block_type=constant  block_config=sysgen:Constant_config
  logi_b19 : hdlBasic/Constant  const=-0.6935483870967741326651889721688348799943923950195312500  gui_display_data_type=Fixed-point  arith_type=Signed (2's comp)  n_bits=32  bin_pt=30  preci_type=Double  exp_width=8  frac_width=24  explicit_period=on  period=1  XmcBlockStatus=1  maskContainerNames=tabcontainer1  block_type=constant  block_config=sysgen:Constant_config
  logi_b2 : hdlBasic/Constant  const=-0.9677419354838709963928522483911365270614624023437500000  gui_display_data_type=Fixed-point  arith_type=Signed (2's comp)  n_bits=32  bin_pt=30  preci_type=Double  exp_width=8  frac_width=24  explicit_period=on  period=1  XmcBlockStatus=1  maskContainerNames=tabcontainer1  block_type=constant  block_config=sysgen:Constant_config
  logi_b20 : hdlBasic/Constant  const=-0.6774193548387096308616150963644031435251235961914062500  gui_display_data_type=Fixed-point  arith_type=Signed (2's comp)  n_bits=32  bin_pt=30  preci_type=Double  exp_width=8  frac_width=24  explicit_period=on  period=1  XmcBlockStatus=1  maskContainerNames=tabcontainer1  block_type=constant  block_config=sysgen:Constant_config
  logi_b21 : hdlBasic/Constant  const=-0.6612903225806451290580412205599714070558547973632812500  gui_display_data_type=Fixed-point  arith_type=Signed (2's comp)  n_bits=32  bin_pt=30  preci_type=Double  exp_width=8  frac_width=24  explicit_period=on  period=1  XmcBlockStatus=1  maskContainerNames=tabcontainer1  block_type=constant  block_config=sysgen:Constant_config
  logi_b22 : hdlBasic/Constant  const=-0.6451612903225806272544673447555396705865859985351562500  gui_display_data_type=Fixed-point  arith_type=Signed (2's comp)  n_bits=32  bin_pt=30  preci_type=Double  exp_width=8  frac_width=24  explicit_period=on  period=1  XmcBlockStatus=1  maskContainerNames=tabcontainer1  block_type=constant  block_config=sysgen:Constant_config
  logi_b23 : hdlBasic/Constant  const=-0.6290322580645161254508934689511079341173171997070312500  gui_display_data_type=Fixed-point  arith_type=Signed (2's comp)  n_bits=32  bin_pt=30  preci_type=Double  exp_width=8  frac_width=24  explicit_period=on  period=1  XmcBlockStatus=1  maskContainerNames=tabcontainer1  block_type=constant  block_config=sysgen:Constant_config
  logi_b24 : hdlBasic/Constant  const=-0.6129032258064516236473195931466761976480484008789062500  gui_display_data_type=Fixed-point  arith_type=Signed (2's comp)  n_bits=32  bin_pt=30  preci_type=Double  exp_width=8  frac_width=24  explicit_period=on  period=1  XmcBlockStatus=1  maskContainerNames=tabcontainer1  block_type=constant  block_config=sysgen:Constant_config
  logi_b25 : hdlBasic/Constant  const=-0.5967741935483871218437457173422444611787796020507812500  gui_display_data_type=Fixed-point  arith_type=Signed (2's comp)  n_bits=32  bin_pt=30  preci_type=Double  exp_width=8  frac_width=24  explicit_period=on  period=1  XmcBlockStatus=1  maskContainerNames=tabcontainer1  block_type=constant  block_config=sysgen:Constant_config
  logi_b26 : hdlBasic/Constant  const=-0.5806451612903225090178693790221586823463439941406250000  gui_display_data_type=Fixed-point  arith_type=Signed (2's comp)  n_bits=32  bin_pt=30  preci_type=Double  exp_width=8  frac_width=24  explicit_period=on  period=1  XmcBlockStatus=1  maskContainerNames=tabcontainer1  block_type=constant  block_config=sysgen:Constant_config
  logi_b27 : hdlBasic/Constant  const=-0.5645161290322580072142955032177269458770751953125000000  gui_display_data_type=Fixed-point  arith_type=Signed (2's comp)  n_bits=32  bin_pt=30  preci_type=Double  exp_width=8  frac_width=24  explicit_period=on  period=1  XmcBlockStatus=1  maskContainerNames=tabcontainer1  block_type=constant  block_config=sysgen:Constant_config
  logi_b28 : hdlBasic/Constant  const=-0.5483870967741935054107216274132952094078063964843750000  gui_display_data_type=Fixed-point  arith_type=Signed (2's comp)  n_bits=32  bin_pt=30  preci_type=Double  exp_width=8  frac_width=24  explicit_period=on  period=1  XmcBlockStatus=1  maskContainerNames=tabcontainer1  block_type=constant  block_config=sysgen:Constant_config
  logi_b29 : hdlBasic/Constant  const=-0.5322580645161290036071477516088634729385375976562500000  gui_display_data_type=Fixed-point  arith_type=Signed (2's comp)  n_bits=32  bin_pt=30  preci_type=Double  exp_width=8  frac_width=24  explicit_period=on  period=1  XmcBlockStatus=1  maskContainerNames=tabcontainer1  block_type=constant  block_config=sysgen:Constant_config
  logi_b3 : hdlBasic/Constant  const=-0.9516129032258063835669759100710507482290267944335937500  gui_display_data_type=Fixed-point  arith_type=Signed (2's comp)  n_bits=32  bin_pt=30  preci_type=Double  exp_width=8  frac_width=24  explicit_period=on  period=1  XmcBlockStatus=1  maskContainerNames=tabcontainer1  block_type=constant  block_config=sysgen:Constant_config
  logi_b30 : hdlBasic/Constant  const=-0.5161290322580645018035738758044317364692687988281250000  gui_display_data_type=Fixed-point  arith_type=Signed (2's comp)  n_bits=32  bin_pt=30  preci_type=Double  exp_width=8  frac_width=24  explicit_period=on  period=1  XmcBlockStatus=1  maskContainerNames=tabcontainer1  block_type=constant  block_config=sysgen:Constant_config
  logi_b31 : hdlBasic/Constant  const=-0.5000000000000000000000000000000000000000000000000000000  gui_display_data_type=Fixed-point  arith_type=Signed (2's comp)  n_bits=32  bin_pt=30  preci_type=Double  exp_width=8  frac_width=24  explicit_period=on  period=1  XmcBlockStatus=1  maskContainerNames=tabcontainer1  block_type=constant  block_config=sysgen:Constant_config
  logi_b32 : hdlBasic/Constant  const=-0.4838709677419354981964261241955682635307312011718750000  gui_display_data_type=Fixed-point  arith_type=Signed (2's comp)  n_bits=32  bin_pt=30  preci_type=Double  exp_width=8  frac_width=24  explicit_period=on  period=1  XmcBlockStatus=1  maskContainerNames=tabcontainer1  block_type=constant  block_config=sysgen:Constant_config
  logi_b33 : hdlBasic/Constant  const=-0.4677419354838709408817010171333095058798789978027343750  gui_display_data_type=Fixed-point  arith_type=Signed (2's comp)  n_bits=32  bin_pt=30  preci_type=Double  exp_width=8  frac_width=24  explicit_period=on  period=1  XmcBlockStatus=1  maskContainerNames=tabcontainer1  block_type=constant  block_config=sysgen:Constant_config
  logi_b34 : hdlBasic/Constant  const=-0.4516129032258064390781271413288777694106101989746093750  gui_display_data_type=Fixed-point  arith_type=Signed (2's comp)  n_bits=32  bin_pt=30  preci_type=Double  exp_width=8  frac_width=24  explicit_period=on  period=1  XmcBlockStatus=1  maskContainerNames=tabcontainer1  block_type=constant  block_config=sysgen:Constant_config
  logi_b35 : hdlBasic/Constant  const=-0.4354838709677419372745532655244460329413414001464843750  gui_display_data_type=Fixed-point  arith_type=Signed (2's comp)  n_bits=32  bin_pt=30  preci_type=Double  exp_width=8  frac_width=24  explicit_period=on  period=1  XmcBlockStatus=1  maskContainerNames=tabcontainer1  block_type=constant  block_config=sysgen:Constant_config
  logi_b36 : hdlBasic/Constant  const=-0.4193548387096773799598281584621872752904891967773437500  gui_display_data_type=Fixed-point  arith_type=Signed (2's comp)  n_bits=32  bin_pt=30  preci_type=Double  exp_width=8  frac_width=24  explicit_period=on  period=1  XmcBlockStatus=1  maskContainerNames=tabcontainer1  block_type=constant  block_config=sysgen:Constant_config
  logi_b37 : hdlBasic/Constant  const=-0.4032258064516128781562542826577555388212203979492187500  gui_display_data_type=Fixed-point  arith_type=Signed (2's comp)  n_bits=32  bin_pt=30  preci_type=Double  exp_width=8  frac_width=24  explicit_period=on  period=1  XmcBlockStatus=1  maskContainerNames=tabcontainer1  block_type=constant  block_config=sysgen:Constant_config
  logi_b38 : hdlBasic/Constant  const=-0.3870967741935483763526804068533238023519515991210937500  gui_display_data_type=Fixed-point  arith_type=Signed (2's comp)  n_bits=32  bin_pt=30  preci_type=Double  exp_width=8  frac_width=24  explicit_period=on  period=1  XmcBlockStatus=1  maskContainerNames=tabcontainer1  block_type=constant  block_config=sysgen:Constant_config
  logi_b39 : hdlBasic/Constant  const=-0.3709677419354838745491065310488920658826828002929687500  gui_display_data_type=Fixed-point  arith_type=Signed (2's comp)  n_bits=32  bin_pt=30  preci_type=Double  exp_width=8  frac_width=24  explicit_period=on  period=1  XmcBlockStatus=1  maskContainerNames=tabcontainer1  block_type=constant  block_config=sysgen:Constant_config
  logi_b4 : hdlBasic/Constant  const=-0.9354838709677418817634020342666190117597579956054687500  gui_display_data_type=Fixed-point  arith_type=Signed (2's comp)  n_bits=32  bin_pt=30  preci_type=Double  exp_width=8  frac_width=24  explicit_period=on  period=1  XmcBlockStatus=1  maskContainerNames=tabcontainer1  block_type=constant  block_config=sysgen:Constant_config
  logi_b40 : hdlBasic/Constant  const=-0.3548387096774193727455326552444603294134140014648437500  gui_display_data_type=Fixed-point  arith_type=Signed (2's comp)  n_bits=32  bin_pt=30  preci_type=Double  exp_width=8  frac_width=24  explicit_period=on  period=1  XmcBlockStatus=1  maskContainerNames=tabcontainer1  block_type=constant  block_config=sysgen:Constant_config
  logi_b41 : hdlBasic/Constant  const=-0.3387096774193548154308075481822015717625617980957031250  gui_display_data_type=Fixed-point  arith_type=Signed (2's comp)  n_bits=32  bin_pt=30  preci_type=Double  exp_width=8  frac_width=24  explicit_period=on  period=1  XmcBlockStatus=1  maskContainerNames=tabcontainer1  block_type=constant  block_config=sysgen:Constant_config
  logi_b42 : hdlBasic/Constant  const=-0.3225806451612903136272336723777698352932929992675781250  gui_display_data_type=Fixed-point  arith_type=Signed (2's comp)  n_bits=32  bin_pt=30  preci_type=Double  exp_width=8  frac_width=24  explicit_period=on  period=1  XmcBlockStatus=1  maskContainerNames=tabcontainer1  block_type=constant  block_config=sysgen:Constant_config
  logi_b43 : hdlBasic/Constant  const=-0.3064516129032258118236597965733380988240242004394531250  gui_display_data_type=Fixed-point  arith_type=Signed (2's comp)  n_bits=32  bin_pt=30  preci_type=Double  exp_width=8  frac_width=24  explicit_period=on  period=1  XmcBlockStatus=1  maskContainerNames=tabcontainer1  block_type=constant  block_config=sysgen:Constant_config
  logi_b44 : hdlBasic/Constant  const=-0.2903225806451612545089346895110793411731719970703125000  gui_display_data_type=Fixed-point  arith_type=Signed (2's comp)  n_bits=32  bin_pt=30  preci_type=Double  exp_width=8  frac_width=24  explicit_period=on  period=1  XmcBlockStatus=1  maskContainerNames=tabcontainer1  block_type=constant  block_config=sysgen:Constant_config
  logi_b45 : hdlBasic/Constant  const=-0.2741935483870967527053608137066476047039031982421875000  gui_display_data_type=Fixed-point  arith_type=Signed (2's comp)  n_bits=32  bin_pt=30  preci_type=Double  exp_width=8  frac_width=24  explicit_period=on  period=1  XmcBlockStatus=1  maskContainerNames=tabcontainer1  block_type=constant  block_config=sysgen:Constant_config
  logi_b46 : hdlBasic/Constant  const=-0.2580645161290322509017869379022158682346343994140625000  gui_display_data_type=Fixed-point  arith_type=Signed (2's comp)  n_bits=32  bin_pt=30  preci_type=Double  exp_width=8  frac_width=24  explicit_period=on  period=1  XmcBlockStatus=1  maskContainerNames=tabcontainer1  block_type=constant  block_config=sysgen:Constant_config
  logi_b47 : hdlBasic/Constant  const=-0.2419354838709677490982130620977841317653656005859375000  gui_display_data_type=Fixed-point  arith_type=Signed (2's comp)  n_bits=32  bin_pt=30  preci_type=Double  exp_width=8  frac_width=24  explicit_period=on  period=1  XmcBlockStatus=1  maskContainerNames=tabcontainer1  block_type=constant  block_config=sysgen:Constant_config
  logi_b48 : hdlBasic/Constant  const=-0.2258064516129032195390635706644388847053050994873046875  gui_display_data_type=Fixed-point  arith_type=Signed (2's comp)  n_bits=32  bin_pt=30  preci_type=Double  exp_width=8  frac_width=24  explicit_period=on  period=1  XmcBlockStatus=1  maskContainerNames=tabcontainer1  block_type=constant  block_config=sysgen:Constant_config
  logi_b49 : hdlBasic/Constant  const=-0.2096774193548386899799140792310936376452445983886718750  gui_display_data_type=Fixed-point  arith_type=Signed (2's comp)  n_bits=32  bin_pt=30  preci_type=Double  exp_width=8  frac_width=24  explicit_period=on  period=1  XmcBlockStatus=1  maskContainerNames=tabcontainer1  block_type=constant  block_config=sysgen:Constant_config
  logi_b5 : hdlBasic/Constant  const=-0.9193548387096773799598281584621872752904891967773437500  gui_display_data_type=Fixed-point  arith_type=Signed (2's comp)  n_bits=32  bin_pt=30  preci_type=Double  exp_width=8  frac_width=24  explicit_period=on  period=1  XmcBlockStatus=1  maskContainerNames=tabcontainer1  block_type=constant  block_config=sysgen:Constant_config
  logi_b50 : hdlBasic/Constant  const=-0.1935483870967741881763402034266619011759757995605468750  gui_display_data_type=Fixed-point  arith_type=Signed (2's comp)  n_bits=32  bin_pt=30  preci_type=Double  exp_width=8  frac_width=24  explicit_period=on  period=1  XmcBlockStatus=1  maskContainerNames=tabcontainer1  block_type=constant  block_config=sysgen:Constant_config
  logi_b51 : hdlBasic/Constant  const=-0.1774193548387096863727663276222301647067070007324218750  gui_display_data_type=Fixed-point  arith_type=Signed (2's comp)  n_bits=32  bin_pt=30  preci_type=Double  exp_width=8  frac_width=24  explicit_period=on  period=1  XmcBlockStatus=1  maskContainerNames=tabcontainer1  block_type=constant  block_config=sysgen:Constant_config
  logi_b52 : hdlBasic/Constant  const=-0.1612903225806451568136168361888849176466464996337890625  gui_display_data_type=Fixed-point  arith_type=Signed (2's comp)  n_bits=32  bin_pt=30  preci_type=Double  exp_width=8  frac_width=24  explicit_period=on  period=1  XmcBlockStatus=1  maskContainerNames=tabcontainer1  block_type=constant  block_config=sysgen:Constant_config
  logi_b53 : hdlBasic/Constant  const=-0.1451612903225806272544673447555396705865859985351562500  gui_display_data_type=Fixed-point  arith_type=Signed (2's comp)  n_bits=32  bin_pt=30  preci_type=Double  exp_width=8  frac_width=24  explicit_period=on  period=1  XmcBlockStatus=1  maskContainerNames=tabcontainer1  block_type=constant  block_config=sysgen:Constant_config
  logi_b54 : hdlBasic/Constant  const=-0.1290322580645161254508934689511079341173171997070312500  gui_display_data_type=Fixed-point  arith_type=Signed (2's comp)  n_bits=32  bin_pt=30  preci_type=Double  exp_width=8  frac_width=24  explicit_period=on  period=1  XmcBlockStatus=1  maskContainerNames=tabcontainer1  block_type=constant  block_config=sysgen:Constant_config
  logi_b55 : hdlBasic/Constant  const=-0.1129032258064516097695317853322194423526525497436523438  gui_display_data_type=Fixed-point  arith_type=Signed (2's comp)  n_bits=32  bin_pt=30  preci_type=Double  exp_width=8  frac_width=24  explicit_period=on  period=1  XmcBlockStatus=1  maskContainerNames=tabcontainer1  block_type=constant  block_config=sysgen:Constant_config
  logi_b56 : hdlBasic/Constant  const=-0.0967741935483870940881701017133309505879878997802734375  gui_display_data_type=Fixed-point  arith_type=Signed (2's comp)  n_bits=32  bin_pt=30  preci_type=Double  exp_width=8  frac_width=24  explicit_period=on  period=1  XmcBlockStatus=1  maskContainerNames=tabcontainer1  block_type=constant  block_config=sysgen:Constant_config
  logi_b57 : hdlBasic/Constant  const=-0.0806451612903225784068084180944424588233232498168945312  gui_display_data_type=Fixed-point  arith_type=Signed (2's comp)  n_bits=32  bin_pt=30  preci_type=Double  exp_width=8  frac_width=24  explicit_period=on  period=1  XmcBlockStatus=1  maskContainerNames=tabcontainer1  block_type=constant  block_config=sysgen:Constant_config
  logi_b58 : hdlBasic/Constant  const=-0.0645161290322580627254467344755539670586585998535156250  gui_display_data_type=Fixed-point  arith_type=Signed (2's comp)  n_bits=32  bin_pt=30  preci_type=Double  exp_width=8  frac_width=24  explicit_period=on  period=1  XmcBlockStatus=1  maskContainerNames=tabcontainer1  block_type=constant  block_config=sysgen:Constant_config
  logi_b59 : hdlBasic/Constant  const=-0.0483870967741935470440850508566654752939939498901367188  gui_display_data_type=Fixed-point  arith_type=Signed (2's comp)  n_bits=32  bin_pt=30  preci_type=Double  exp_width=8  frac_width=24  explicit_period=on  period=1  XmcBlockStatus=1  maskContainerNames=tabcontainer1  block_type=constant  block_config=sysgen:Constant_config
  logi_b6 : hdlBasic/Constant  const=-0.9032258064516128781562542826577555388212203979492187500  gui_display_data_type=Fixed-point  arith_type=Signed (2's comp)  n_bits=32  bin_pt=30  preci_type=Double  exp_width=8  frac_width=24  explicit_period=on  period=1  XmcBlockStatus=1  maskContainerNames=tabcontainer1  block_type=constant  block_config=sysgen:Constant_config
  logi_b60 : hdlBasic/Constant  const=-0.0322580645161290313627233672377769835293292999267578125  gui_display_data_type=Fixed-point  arith_type=Signed (2's comp)  n_bits=32  bin_pt=30  preci_type=Double  exp_width=8  frac_width=24  explicit_period=on  period=1  XmcBlockStatus=1  maskContainerNames=tabcontainer1  block_type=constant  block_config=sysgen:Constant_config
  logi_b61 : hdlBasic/Constant  const=-0.0161290322580645156813616836188884917646646499633789062  gui_display_data_type=Fixed-point  arith_type=Signed (2's comp)  n_bits=32  bin_pt=30  preci_type=Double  exp_width=8  frac_width=24  explicit_period=on  period=1  XmcBlockStatus=1  maskContainerNames=tabcontainer1  block_type=constant  block_config=sysgen:Constant_config
  logi_b62 : hdlBasic/Constant  const=0.0000000000000000000000000000000000000000000000000000000  gui_display_data_type=Fixed-point  arith_type=Signed (2's comp)  n_bits=32  bin_pt=30  preci_type=Double  exp_width=8  frac_width=24  explicit_period=on  period=1  XmcBlockStatus=1  maskContainerNames=tabcontainer1  block_type=constant  block_config=sysgen:Constant_config
  logi_b63 : hdlBasic/Constant  const=0.0161290322580645156813616836188884917646646499633789062  gui_display_data_type=Fixed-point  arith_type=Signed (2's comp)  n_bits=32  bin_pt=30  preci_type=Double  exp_width=8  frac_width=24  explicit_period=on  period=1  XmcBlockStatus=1  maskContainerNames=tabcontainer1  block_type=constant  block_config=sysgen:Constant_config
  logi_b64 : hdlBasic/Constant  const=0.0322580645161290313627233672377769835293292999267578125  gui_display_data_type=Fixed-point  arith_type=Signed (2's comp)  n_bits=32  bin_pt=30  preci_type=Double  exp_width=8  frac_width=24  explicit_period=on  period=1  XmcBlockStatus=1  maskContainerNames=tabcontainer1  block_type=constant  block_config=sysgen:Constant_config
  logi_b65 : hdlBasic/Constant  const=0.0483870967741935470440850508566654752939939498901367188  gui_display_data_type=Fixed-point  arith_type=Signed (2's comp)  n_bits=32  bin_pt=30  preci_type=Double  exp_width=8  frac_width=24  explicit_period=on  period=1  XmcBlockStatus=1  maskContainerNames=tabcontainer1  block_type=constant  block_config=sysgen:Constant_config
  logi_b66 : hdlBasic/Constant  const=0.0645161290322580627254467344755539670586585998535156250  gui_display_data_type=Fixed-point  arith_type=Signed (2's comp)  n_bits=32  bin_pt=30  preci_type=Double  exp_width=8  frac_width=24  explicit_period=on  period=1  XmcBlockStatus=1  maskContainerNames=tabcontainer1  block_type=constant  block_config=sysgen:Constant_config
  logi_b67 : hdlBasic/Constant  const=0.0806451612903225784068084180944424588233232498168945312  gui_display_data_type=Fixed-point  arith_type=Signed (2's comp)  n_bits=32  bin_pt=30  preci_type=Double  exp_width=8  frac_width=24  explicit_period=on  period=1  XmcBlockStatus=1  maskContainerNames=tabcontainer1  block_type=constant  block_config=sysgen:Constant_config
  logi_b68 : hdlBasic/Constant  const=0.0967741935483870940881701017133309505879878997802734375  gui_display_data_type=Fixed-point  arith_type=Signed (2's comp)  n_bits=32  bin_pt=30  preci_type=Double  exp_width=8  frac_width=24  explicit_period=on  period=1  XmcBlockStatus=1  maskContainerNames=tabcontainer1  block_type=constant  block_config=sysgen:Constant_config
  logi_b69 : hdlBasic/Constant  const=0.1129032258064516097695317853322194423526525497436523438  gui_display_data_type=Fixed-point  arith_type=Signed (2's comp)  n_bits=32  bin_pt=30  preci_type=Double  exp_width=8  frac_width=24  explicit_period=on  period=1  XmcBlockStatus=1  maskContainerNames=tabcontainer1  block_type=constant  block_config=sysgen:Constant_config
  logi_b7 : hdlBasic/Constant  const=-0.8870967741935483763526804068533238023519515991210937500  gui_display_data_type=Fixed-point  arith_type=Signed (2's comp)  n_bits=32  bin_pt=30  preci_type=Double  exp_width=8  frac_width=24  explicit_period=on  period=1  XmcBlockStatus=1  maskContainerNames=tabcontainer1  block_type=constant  block_config=sysgen:Constant_config
  logi_b70 : hdlBasic/Constant  const=0.1290322580645161254508934689511079341173171997070312500  gui_display_data_type=Fixed-point  arith_type=Signed (2's comp)  n_bits=32  bin_pt=30  preci_type=Double  exp_width=8  frac_width=24  explicit_period=on  period=1  XmcBlockStatus=1  maskContainerNames=tabcontainer1  block_type=constant  block_config=sysgen:Constant_config
  logi_b71 : hdlBasic/Constant  const=0.1451612903225806272544673447555396705865859985351562500  gui_display_data_type=Fixed-point  arith_type=Signed (2's comp)  n_bits=32  bin_pt=30  preci_type=Double  exp_width=8  frac_width=24  explicit_period=on  period=1  XmcBlockStatus=1  maskContainerNames=tabcontainer1  block_type=constant  block_config=sysgen:Constant_config
  logi_b72 : hdlBasic/Constant  const=0.1612903225806451568136168361888849176466464996337890625  gui_display_data_type=Fixed-point  arith_type=Signed (2's comp)  n_bits=32  bin_pt=30  preci_type=Double  exp_width=8  frac_width=24  explicit_period=on  period=1  XmcBlockStatus=1  maskContainerNames=tabcontainer1  block_type=constant  block_config=sysgen:Constant_config
  logi_b73 : hdlBasic/Constant  const=0.1774193548387096863727663276222301647067070007324218750  gui_display_data_type=Fixed-point  arith_type=Signed (2's comp)  n_bits=32  bin_pt=30  preci_type=Double  exp_width=8  frac_width=24  explicit_period=on  period=1  XmcBlockStatus=1  maskContainerNames=tabcontainer1  block_type=constant  block_config=sysgen:Constant_config
  logi_b74 : hdlBasic/Constant  const=0.1935483870967741881763402034266619011759757995605468750  gui_display_data_type=Fixed-point  arith_type=Signed (2's comp)  n_bits=32  bin_pt=30  preci_type=Double  exp_width=8  frac_width=24  explicit_period=on  period=1  XmcBlockStatus=1  maskContainerNames=tabcontainer1  block_type=constant  block_config=sysgen:Constant_config
  logi_b75 : hdlBasic/Constant  const=0.2096774193548386899799140792310936376452445983886718750  gui_display_data_type=Fixed-point  arith_type=Signed (2's comp)  n_bits=32  bin_pt=30  preci_type=Double  exp_width=8  frac_width=24  explicit_period=on  period=1  XmcBlockStatus=1  maskContainerNames=tabcontainer1  block_type=constant  block_config=sysgen:Constant_config
  logi_b76 : hdlBasic/Constant  const=0.2258064516129032195390635706644388847053050994873046875  gui_display_data_type=Fixed-point  arith_type=Signed (2's comp)  n_bits=32  bin_pt=30  preci_type=Double  exp_width=8  frac_width=24  explicit_period=on  period=1  XmcBlockStatus=1  maskContainerNames=tabcontainer1  block_type=constant  block_config=sysgen:Constant_config
  logi_b77 : hdlBasic/Constant  const=0.2419354838709677490982130620977841317653656005859375000  gui_display_data_type=Fixed-point  arith_type=Signed (2's comp)  n_bits=32  bin_pt=30  preci_type=Double  exp_width=8  frac_width=24  explicit_period=on  period=1  XmcBlockStatus=1  maskContainerNames=tabcontainer1  block_type=constant  block_config=sysgen:Constant_config
  logi_b78 : hdlBasic/Constant  const=0.2580645161290322509017869379022158682346343994140625000  gui_display_data_type=Fixed-point  arith_type=Signed (2's comp)  n_bits=32  bin_pt=30  preci_type=Double  exp_width=8  frac_width=24  explicit_period=on  period=1  XmcBlockStatus=1  maskContainerNames=tabcontainer1  block_type=constant  block_config=sysgen:Constant_config
  logi_b79 : hdlBasic/Constant  const=0.2741935483870967527053608137066476047039031982421875000  gui_display_data_type=Fixed-point  arith_type=Signed (2's comp)  n_bits=32  bin_pt=30  preci_type=Double  exp_width=8  frac_width=24  explicit_period=on  period=1  XmcBlockStatus=1  maskContainerNames=tabcontainer1  block_type=constant  block_config=sysgen:Constant_config
  logi_b8 : hdlBasic/Constant  const=-0.8709677419354838745491065310488920658826828002929687500  gui_display_data_type=Fixed-point  arith_type=Signed (2's comp)  n_bits=32  bin_pt=30  preci_type=Double  exp_width=8  frac_width=24  explicit_period=on  period=1  XmcBlockStatus=1  maskContainerNames=tabcontainer1  block_type=constant  block_config=sysgen:Constant_config
  logi_b80 : hdlBasic/Constant  const=0.2903225806451612545089346895110793411731719970703125000  gui_display_data_type=Fixed-point  arith_type=Signed (2's comp)  n_bits=32  bin_pt=30  preci_type=Double  exp_width=8  frac_width=24  explicit_period=on  period=1  XmcBlockStatus=1  maskContainerNames=tabcontainer1  block_type=constant  block_config=sysgen:Constant_config
  logi_b81 : hdlBasic/Constant  const=0.3064516129032258118236597965733380988240242004394531250  gui_display_data_type=Fixed-point  arith_type=Signed (2's comp)  n_bits=32  bin_pt=30  preci_type=Double  exp_width=8  frac_width=24  explicit_period=on  period=1  XmcBlockStatus=1  maskContainerNames=tabcontainer1  block_type=constant  block_config=sysgen:Constant_config
  logi_b82 : hdlBasic/Constant  const=0.3225806451612903136272336723777698352932929992675781250  gui_display_data_type=Fixed-point  arith_type=Signed (2's comp)  n_bits=32  bin_pt=30  preci_type=Double  exp_width=8  frac_width=24  explicit_period=on  period=1  XmcBlockStatus=1  maskContainerNames=tabcontainer1  block_type=constant  block_config=sysgen:Constant_config
  logi_b83 : hdlBasic/Constant  const=0.3387096774193548154308075481822015717625617980957031250  gui_display_data_type=Fixed-point  arith_type=Signed (2's comp)  n_bits=32  bin_pt=30  preci_type=Double  exp_width=8  frac_width=24  explicit_period=on  period=1  XmcBlockStatus=1  maskContainerNames=tabcontainer1  block_type=constant  block_config=sysgen:Constant_config
  logi_b84 : hdlBasic/Constant  const=0.3548387096774193727455326552444603294134140014648437500  gui_display_data_type=Fixed-point  arith_type=Signed (2's comp)  n_bits=32  bin_pt=30  preci_type=Double  exp_width=8  frac_width=24  explicit_period=on  period=1  XmcBlockStatus=1  maskContainerNames=tabcontainer1  block_type=constant  block_config=sysgen:Constant_config
  logi_b85 : hdlBasic/Constant  const=0.3709677419354838745491065310488920658826828002929687500  gui_display_data_type=Fixed-point  arith_type=Signed (2's comp)  n_bits=32  bin_pt=30  preci_type=Double  exp_width=8  frac_width=24  explicit_period=on  period=1  XmcBlockStatus=1  maskContainerNames=tabcontainer1  block_type=constant  block_config=sysgen:Constant_config
  logi_b86 : hdlBasic/Constant  const=0.3870967741935483763526804068533238023519515991210937500  gui_display_data_type=Fixed-point  arith_type=Signed (2's comp)  n_bits=32  bin_pt=30  preci_type=Double  exp_width=8  frac_width=24  explicit_period=on  period=1  XmcBlockStatus=1  maskContainerNames=tabcontainer1  block_type=constant  block_config=sysgen:Constant_config
  logi_b87 : hdlBasic/Constant  const=0.4032258064516128781562542826577555388212203979492187500  gui_display_data_type=Fixed-point  arith_type=Signed (2's comp)  n_bits=32  bin_pt=30  preci_type=Double  exp_width=8  frac_width=24  explicit_period=on  period=1  XmcBlockStatus=1  maskContainerNames=tabcontainer1  block_type=constant  block_config=sysgen:Constant_config
  logi_b88 : hdlBasic/Constant  const=0.4193548387096773799598281584621872752904891967773437500  gui_display_data_type=Fixed-point  arith_type=Signed (2's comp)  n_bits=32  bin_pt=30  preci_type=Double  exp_width=8  frac_width=24  explicit_period=on  period=1  XmcBlockStatus=1  maskContainerNames=tabcontainer1  block_type=constant  block_config=sysgen:Constant_config
  logi_b89 : hdlBasic/Constant  const=0.4354838709677419372745532655244460329413414001464843750  gui_display_data_type=Fixed-point  arith_type=Signed (2's comp)  n_bits=32  bin_pt=30  preci_type=Double  exp_width=8  frac_width=24  explicit_period=on  period=1  XmcBlockStatus=1  maskContainerNames=tabcontainer1  block_type=constant  block_config=sysgen:Constant_config
  logi_b9 : hdlBasic/Constant  const=-0.8548387096774193727455326552444603294134140014648437500  gui_display_data_type=Fixed-point  arith_type=Signed (2's comp)  n_bits=32  bin_pt=30  preci_type=Double  exp_width=8  frac_width=24  explicit_period=on  period=1  XmcBlockStatus=1  maskContainerNames=tabcontainer1  block_type=constant  block_config=sysgen:Constant_config
  logi_b90 : hdlBasic/Constant  const=0.4516129032258064390781271413288777694106101989746093750  gui_display_data_type=Fixed-point  arith_type=Signed (2's comp)  n_bits=32  bin_pt=30  preci_type=Double  exp_width=8  frac_width=24  explicit_period=on  period=1  XmcBlockStatus=1  maskContainerNames=tabcontainer1  block_type=constant  block_config=sysgen:Constant_config
  logi_b91 : hdlBasic/Constant  const=0.4677419354838709408817010171333095058798789978027343750  gui_display_data_type=Fixed-point  arith_type=Signed (2's comp)  n_bits=32  bin_pt=30  preci_type=Double  exp_width=8  frac_width=24  explicit_period=on  period=1  XmcBlockStatus=1  maskContainerNames=tabcontainer1  block_type=constant  block_config=sysgen:Constant_config
  logi_b92 : hdlBasic/Constant  const=0.4838709677419354981964261241955682635307312011718750000  gui_display_data_type=Fixed-point  arith_type=Signed (2's comp)  n_bits=32  bin_pt=30  preci_type=Double  exp_width=8  frac_width=24  explicit_period=on  period=1  XmcBlockStatus=1  maskContainerNames=tabcontainer1  block_type=constant  block_config=sysgen:Constant_config
  logi_b93 : hdlBasic/Constant  const=0.5000000000000000000000000000000000000000000000000000000  gui_display_data_type=Fixed-point  arith_type=Signed (2's comp)  n_bits=32  bin_pt=30  preci_type=Double  exp_width=8  frac_width=24  explicit_period=on  period=1  XmcBlockStatus=1  maskContainerNames=tabcontainer1  block_type=constant  block_config=sysgen:Constant_config
  logi_b94 : hdlBasic/Constant  const=0.5161290322580645018035738758044317364692687988281250000  gui_display_data_type=Fixed-point  arith_type=Signed (2's comp)  n_bits=32  bin_pt=30  preci_type=Double  exp_width=8  frac_width=24  explicit_period=on  period=1  XmcBlockStatus=1  maskContainerNames=tabcontainer1  block_type=constant  block_config=sysgen:Constant_config
  logi_b95 : hdlBasic/Constant  const=0.5322580645161290036071477516088634729385375976562500000  gui_display_data_type=Fixed-point  arith_type=Signed (2's comp)  n_bits=32  bin_pt=30  preci_type=Double  exp_width=8  frac_width=24  explicit_period=on  period=1  XmcBlockStatus=1  maskContainerNames=tabcontainer1  block_type=constant  block_config=sysgen:Constant_config
  logi_b96 : hdlBasic/Constant  const=0.5483870967741935054107216274132952094078063964843750000  gui_display_data_type=Fixed-point  arith_type=Signed (2's comp)  n_bits=32  bin_pt=30  preci_type=Double  exp_width=8  frac_width=24  explicit_period=on  period=1  XmcBlockStatus=1  maskContainerNames=tabcontainer1  block_type=constant  block_config=sysgen:Constant_config
  logi_b97 : hdlBasic/Constant  const=0.5645161290322580072142955032177269458770751953125000000  gui_display_data_type=Fixed-point  arith_type=Signed (2's comp)  n_bits=32  bin_pt=30  preci_type=Double  exp_width=8  frac_width=24  explicit_period=on  period=1  XmcBlockStatus=1  maskContainerNames=tabcontainer1  block_type=constant  block_config=sysgen:Constant_config
  logi_b98 : hdlBasic/Constant  const=0.5806451612903225090178693790221586823463439941406250000  gui_display_data_type=Fixed-point  arith_type=Signed (2's comp)  n_bits=32  bin_pt=30  preci_type=Double  exp_width=8  frac_width=24  explicit_period=on  period=1  XmcBlockStatus=1  maskContainerNames=tabcontainer1  block_type=constant  block_config=sysgen:Constant_config
  logi_b99 : hdlBasic/Constant  const=0.5967741935483871218437457173422444611787796020507812500  gui_display_data_type=Fixed-point  arith_type=Signed (2's comp)  n_bits=32  bin_pt=30  preci_type=Double  exp_width=8  frac_width=24  explicit_period=on  period=1  XmcBlockStatus=1  maskContainerNames=tabcontainer1  block_type=constant  block_config=sysgen:Constant_config
  logical_x0 : hdlBasic/Mux  inputs=2  en=off  latency=1  precision=Full  arith_type=Unsigned  n_bits=16  bin_pt=14  quantization=Truncate  overflow=Wrap  XmcBlockStatus=1  maskContainerNames=tabcontainer1  block_type=mux  block_config=sysgen:Mux_config
  logical_y0 : hdlBasic/Mux  inputs=2  en=off  latency=1  precision=Full  arith_type=Unsigned  n_bits=16  bin_pt=14  quantization=Truncate  overflow=Wrap  XmcBlockStatus=1  maskContainerNames=tabcontainer1  block_type=mux  block_config=sysgen:Mux_config
  Output : Outport
  wires:
  Mux1/1 -> AddSub1/1, Delay10/1
  AddSub4/1 -> Mux5/3
  In4/1 -> Gate_In2/1
  Mux3/1 -> AddSub3/1, Delay16/1
  Relational3/1 -> Delay9/1
  Mux2/1 -> AddSub2/1, Delay13/1
  Gate_In2/1 -> Relational/2, Delay3/1, Delay2/1
  Mux6/1 -> AddSub6/1, Delay26/1
  AddSub6/1 -> Mux7/3
  In3/1 -> Gate_In1/1
  AddSub/1 -> Mux1/3
  Relational6/1 -> Delay19/1
  AddSub2/1 -> Mux3/3
  Mux/1 -> Delay7/1, AddSub/1
  AddSub1/1 -> Mux2/3
  Relational7/1 -> Delay22/1
  Mux4/1 -> AddSub4/1, Delay20/1
  Relational2/1 -> Mux/1
  AddSub3/1 -> Mux4/3
  Mux7/1 -> AddSub7/1, Delay29/1
  Relational5/1 -> Delay15/1
  Relational4/1 -> Delay12/1
  AddSub5/1 -> Mux6/3
  Mux5/1 -> AddSub5/1, Delay23/1
  AddSub7/1 -> Mux8/3
  Relational8/1 -> Delay25/1
  Gate_In1/1 -> Relational/1, Delay4/1, Delay1/1
  Relational1/1 -> Delay6/1
  Relational9/1 -> Delay28/1
  logical_y0/1 -> Relational2/1, Delay5/1
  Relational/1 -> logical_x0/1, logical_y0/1
  Constant3/1 -> AddSub19/2
  Constant/1 -> AddSub18/2
  AddSub19/1 -> Mult/2
  AddSub18/1 -> Negate/1
  Constant4/1 -> Mult1/2
  AddSub22/1 -> Slice3/1
  AddSub21/1 -> AddSub22/1
  AddSub20/1 -> AddSub21/1
  Mult1/1 -> AddSub20/1
  Negate/1 -> AddSub19/1
  Mult/1 -> Slice2/1
  Delay1/1 -> logical_y0/2
  Delay2/1 -> logical_y0/3
  Delay3/1 -> logical_x0/2
  Delay4/1 -> logical_x0/3
  Delay5/1 -> Relational1/1, Delay8/1
  Delay6/1 -> Mux1/1
  Delay7/1 -> Mux1/2
  Delay8/1 -> Relational3/1, Delay11/1
  Delay9/1 -> Mux2/1
  Delay10/1 -> Mux2/2
  Delay11/1 -> Relational4/1, Delay14/1
  Delay12/1 -> Mux3/1
  Delay13/1 -> Mux3/2
  Delay14/1 -> Relational5/1, Delay17/1
  Delay15/1 -> Mux4/1
  Delay16/1 -> Mux4/2
  Delay17/1 -> Delay18/1, Relational6/1
  Delay18/1 -> Delay21/1, Relational7/1
  Delay19/1 -> Mux5/1
  Delay20/1 -> Mux5/2
  Delay21/1 -> Delay24/1, Relational8/1
  Delay22/1 -> Mux6/1
  Delay23/1 -> Mux6/2
  Delay24/1 -> Relational9/1, Delay27/1
  Delay25/1 -> Mux7/1
  Delay26/1 -> Mux7/2
  Delay28/1 -> Mux8/1
  Delay29/1 -> Mux8/2
  Delay32/1 -> Mux22/2
  Delay48/1 -> Mux27/2
  Relational30/1 -> Delay50/1
  Delay50/1 -> Mux28/1
  Delay36/1 -> Relational26/1, Delay39/1
  Mux24/1 -> AddSub27/1, Delay42/1
  Delay37/1 -> Mux24/1
  logi_b3/1 -> Relational25/2, Relational4/2
  AddSub24/1 -> Mux22/3
  AddSub28/1 -> Mux26/3
  Delay46/1 -> Relational30/1, Delay49/1
  Delay54/1 -> Delay57/1, Relational21/1
  Delay41/1 -> Mux25/1
  logi_b1/1 -> Relational21/2, Relational1/2
  Relational23/1 -> Mux20/1
  AddSub25/1 -> Mux23/3
  Delay35/1 -> Mux23/2
  Delay44/1 -> Mux26/1
  Relational27/1 -> Delay41/1
  logi_b4/1 -> Relational26/2, Relational5/2
  Delay38/1 -> Mux24/2
  logi_b7/1 -> Relational29/2, Relational8/2
  Delay47/1 -> Mux27/1
  Relational24/1 -> Delay58/1
  logi_b0/1 -> Relational23/2, Relational2/2
  Delay51/1 -> Mux28/2
  Delay57/1 -> Delay33/1, Relational24/1
  logi_b5/1 -> Relational27/2, Relational6/2
  Delay56/1 -> Mux21/2
  Delay34/1 -> Mux23/1
  Mux21/1 -> AddSub24/1, Delay32/1
  Relational21/1 -> Delay55/1
  Delay33/1 -> Relational25/1, Delay36/1
  Delay40/1 -> Delay43/1, Relational28/1
  Delay45/1 -> Mux26/2
  Delay43/1 -> Delay46/1, Relational29/1
  Delay58/1 -> Mux22/1
  logi_b2/1 -> Relational3/2, Relational24/2
  AddSub26/1 -> Mux24/3
  Mux22/1 -> AddSub25/1, Delay35/1
  AddSub29/1 -> Mux27/3
  Relational26/1 -> Delay37/1
  Delay42/1 -> Mux25/2
  logi_b6/1 -> Relational28/2, Relational7/2
  Delay55/1 -> Mux21/1
  Delay39/1 -> Delay40/1, Relational27/1
  Mux23/1 -> AddSub26/1, Delay38/1
  Mux20/1 -> Delay56/1, AddSub23/1
  Mux25/1 -> AddSub28/1, Delay45/1
  Mux27/1 -> AddSub30/1, Delay51/1
  Relational29/1 -> Delay47/1
  AddSub27/1 -> Mux25/3
  AddSub30/1 -> Mux28/3
  Relational28/1 -> Delay44/1
  logi_b8/1 -> Relational30/2, Relational9/2
  AddSub23/1 -> Mux21/3
  Mux26/1 -> AddSub29/1, Delay48/1
  logical_x0/1 -> Relational23/1, Delay54/1
  Constant6/1 -> Mux20/2
  Relational25/1 -> Delay34/1
  Constant1/1 -> Mux/2
  Delay59/1 -> Mult1/1
  Delay60/1 -> Mult/1
  Delay61/1 -> AddSub21/2
  Delay100/1 -> Mux31/1
  Delay94/1 -> Mux19/1
  Delay75/1 -> Mux35/2
  Delay87/1 -> Mux17/1
  Delay73/1 -> Delay76/1, Relational35/1
  Delay91/1 -> Mux18/1
  Mux32/1 -> AddSub33/1, Delay68/1
  Delay92/1 -> Mux18/2
  Relational18/1 -> Delay97/1
  AddSub16/1 -> Mux18/3
  Mux12/1 -> AddSub11/1, Delay65/1
  Delay105/1 -> Mux15/1
  Relational14/1 -> Delay84/1
  Delay85/1 -> Mux16/2
  Delay104/1 -> Delay83/1, Relational13/1
  Delay93/1 -> Delay96/1, Relational18/1
  Mux29/1 -> Delay107/1, AddSub9/1
  Relational13/1 -> Delay105/1
  Mux15/1 -> AddSub14/1, Delay85/1
  Relational12/1 -> Delay102/1
  Mux18/1 -> AddSub17/1, Delay95/1
  AddSub9/1 -> Mux11/3
  Delay96/1 -> Relational20/1, Delay99/1
  AddSub33/1 -> Mux33/3
  Delay108/1 -> Delay63/1, Relational19/1
  Relational19/1 -> Delay109/1
  Mux30/1 -> AddSub34/1, Delay101/1
  logi_b11/1 -> Relational13/2, Relational19/2
  Mux11/1 -> AddSub10/1, Delay62/1
  Delay80/1 -> Mux37/1
  Delay71/1 -> Mux34/1
  AddSub32/1 -> Mux30/3
  Delay97/1 -> Mux30/1
  Delay67/1 -> Mux33/1
  Relational16/1 -> Delay91/1
  Relational17/1 -> Delay94/1
  logi_b13/1 -> Relational15/2, Relational32/2
  Delay69/1 -> Delay70/1, Relational33/1
  logi_b15/1 -> Relational17/2, Relational34/2
  Mux19/1 -> AddSub32/1, Delay98/1
  Mux36/1 -> AddSub38/1, Delay81/1
  Relational20/1 -> Delay100/1
  Relational15/1 -> Delay87/1
  Delay76/1 -> Relational36/1, Delay79/1
  Delay84/1 -> Mux16/1
  Mux34/1 -> AddSub36/1, Delay75/1
  AddSub13/1 -> Mux15/3
  logi_b17/1 -> Relational20/2, Relational36/2
  AddSub36/1 -> Mux35/3
  Mux33/1 -> AddSub35/1, Delay72/1
  Mux35/1 -> AddSub37/1, Delay78/1
  Mux17/1 -> AddSub16/1, Delay92/1
  Delay88/1 -> Mux17/2
  Delay66/1 -> Relational32/1, Delay69/1
  AddSub15/1 -> Mux17/3
  Delay89/1 -> Delay90/1, Relational16/1
  Delay109/1 -> Mux12/1
  Delay77/1 -> Mux36/1
  Delay98/1 -> Mux30/2
  AddSub38/1 -> Mux37/3
  Delay72/1 -> Mux34/2
  AddSub35/1 -> Mux34/3
  Mux9/1 -> Delay103/1, AddSub12/1
  AddSub14/1 -> Mux16/3
  Delay95/1 -> Mux19/2
  logi_b12/1 -> Relational14/2, Relational31/2
  Relational34/1 -> Delay74/1
  Delay102/1 -> Mux14/1
  Delay83/1 -> Relational14/1, Delay86/1
  Delay74/1 -> Mux35/1
  Delay81/1 -> Mux37/2
  logi_b10/1 -> Relational12/2, Relational11/2
  logi_b16/1 -> Relational18/2, Relational35/2
  Mux14/1 -> AddSub13/1, Delay82/1
  Delay90/1 -> Delay93/1, Relational17/1
  AddSub12/1 -> Mux14/3
  Relational33/1 -> Delay71/1
  Relational36/1 -> Delay80/1
  Relational11/1 -> Delay106/1
  AddSub34/1 -> Mux31/3
  Delay86/1 -> Relational15/1, Delay89/1
  Delay68/1 -> Mux33/2
  Relational35/1 -> Delay77/1
  Mux16/1 -> AddSub15/1, Delay88/1
  AddSub11/1 -> Mux32/3
  Relational31/1 -> Delay64/1
  Relational32/1 -> Delay67/1
  Delay107/1 -> Mux11/2
  AddSub10/1 -> Mux12/3
  Delay101/1 -> Mux31/2
  Delay103/1 -> Mux14/2
  Delay65/1 -> Mux32/2
  Delay62/1 -> Mux12/2
  AddSub17/1 -> Mux19/3
  AddSub37/1 -> Mux36/3
  Delay70/1 -> Delay73/1, Relational34/1
  logi_b14/1 -> Relational16/2, Relational33/2
  Delay106/1 -> Mux11/1
  Delay82/1 -> Mux15/2
  Delay78/1 -> Mux36/2
  Delay64/1 -> Mux32/1
  Delay63/1 -> Relational31/1, Delay66/1
  Delay111/1 -> Mux39/2
  logi_b49/1 -> Relational38/2, Relational37/2
  Relational37/1 -> Delay110/1
  Delay110/1 -> Mux39/1
  Mux99/1 -> AddSub40/1, Delay111/1
  AddSub39/1 -> Mux38/3
  Delay112/1 -> Mux38/1
  Mux92/1 -> AddSub39/1, Delay113/1
  AddSub40/1 -> Mux39/3
  Relational38/1 -> Delay112/1
  Delay113/1 -> Mux38/2
  AddSub8/1 -> Mux9/3
  AddSub31/1 -> Mux29/3
  Delay49/1 -> Relational10/1, Delay53/1
  Relational10/1 -> Delay114/1
  Delay31/1 -> Mux29/1
  Relational22/1 -> Delay31/1
  Mux28/1 -> AddSub8/1, Delay115/1
  Delay115/1 -> Mux9/2
  Delay52/1 -> Mux29/2
  Delay114/1 -> Mux9/1
  Mux8/1 -> AddSub31/1, Delay52/1
  logi_b9/1 -> Relational10/2, Relational22/2
  Delay27/1 -> Relational22/1, Delay30/1
  AddSub41/1 -> Mux40/3
  AddSub42/1 -> Mux41/3
  Delay99/1 -> Relational39/1, Delay119/1
  Relational39/1 -> Delay120/1
  Delay117/1 -> Mux41/1
  Relational40/1 -> Delay117/1
  Mux31/1 -> AddSub41/1, Delay121/1
  Delay121/1 -> Mux40/2
  Delay118/1 -> Mux41/2
  Delay120/1 -> Mux40/1
  Mux37/1 -> AddSub42/1, Delay118/1
  logi_b18/1 -> Relational39/2, Relational40/2
  Delay79/1 -> Relational40/1, Delay116/1
  Delay30/1 -> Relational11/1, Delay108/1
  Delay53/1 -> Relational12/1, Delay104/1
  Delay116/1 -> Relational41/1, Delay130/1
  Delay154/1 -> Mux54/2
  AddSub50/1 -> Mux47/3
  Delay125/1 -> Mux42/2
  AddSub56/1 -> Mux54/3
  Relational58/1 -> Delay133/1
  Delay123/1 -> Mux49/2
  Mux43/1 -> AddSub47/1, Delay161/1
  Relational42/1 -> Delay124/1
  Delay140/1 -> Mux50/1
  Relational52/1 -> Delay143/1
  Mux53/1 -> AddSub56/1, Delay154/1
  Relational55/1 -> Delay153/1
  Delay144/1 -> Mux51/2
  Relational51/1 -> Delay140/1
  AddSub53/1 -> Mux49/3
  Relational41/1 -> Delay128/1
  Delay145/1 -> Delay146/1, Relational53/1
  logi_b25/1 -> Relational48/2, Relational55/2
  Relational43/1 -> Delay127/1
  Delay142/1 -> Relational52/1, Delay145/1
  Mux45/1 -> AddSub49/1, Delay168/1
  Mux51/1 -> AddSub54/1, Delay148/1
  Delay170/1 -> Mux47/1
  Delay138/1 -> Mux13/2
  Delay162/1 -> Relational45/1, Delay165/1
  logi_b26/1 -> Relational50/2, Relational56/2
  AddSub46/1 -> Mux43/3
  Relational56/1 -> Delay156/1
  Relational53/1 -> Delay147/1
  Delay167/1 -> Mux46/1
  Relational57/1 -> Delay136/1
  Delay130/1 -> Delay139/1, Relational49/1
  Delay134/1 -> Mux57/2
  Delay164/1 -> Mux45/2
  Delay173/1 -> Mux48/1
  AddSub58/1 -> Mux56/3
  Relational45/1 -> Delay163/1
  logi_b22/1 -> Relational45/2, Relational52/2
  Relational50/1 -> Delay122/1
  Relational47/1 -> Delay170/1
  AddSub59/1 -> Mux57/3
  Delay122/1 -> Mux49/1
  Delay137/1 -> Mux56/2
  Relational46/1 -> Delay167/1
  AddSub51/1 -> Mux48/3
  Mux10/1 -> AddSub43/1, Delay138/1
  Delay128/1 -> Mux10/1
  Delay129/1 -> Mux10/2
  AddSub55/1 -> Mux53/3
  Mux54/1 -> AddSub57/1, Delay157/1
  Delay161/1 -> Mux44/2
  logi_b23/1 -> Relational46/2, Relational53/2
  Delay139/1 -> Relational51/1, Delay142/1
  Delay143/1 -> Mux51/1
  Mux48/1 -> AddSub53/1, Delay123/1
  Delay175/1 -> Relational57/1, Delay135/1
  logi_b24/1 -> Relational47/2, Relational54/2
  Mux40/1 -> Delay125/1, AddSub45/1
  AddSub48/1 -> Mux45/3
  Delay168/1 -> Mux46/2
  Delay152/1 -> Relational56/1, Delay155/1
  Mux42/1 -> AddSub46/1, Delay158/1
  AddSub43/1 -> Mux13/3
  Delay133/1 -> Mux57/1
  AddSub52/1 -> Mux51/3
  Delay126/1 -> Delay159/1, Relational43/1
  Mux49/1 -> AddSub58/1, Delay137/1
  AddSub44/1 -> Mux50/3
  Delay165/1 -> Delay166/1, Relational46/1
  Delay147/1 -> Mux52/1
  Mux13/1 -> AddSub44/1, Delay141/1
  AddSub45/1 -> Mux42/3
  logi_b19/1 -> Relational42/2, Relational41/2
  AddSub60/1 -> Mux10/3
  Delay127/1 -> Mux43/1
  Delay166/1 -> Delay169/1, Relational47/1
  logi_b27/1 -> Relational57/2, Relational58/2
  Mux46/1 -> AddSub50/1, Delay171/1
  Delay141/1 -> Mux50/2
  logi_b21/1 -> Relational44/2, Relational51/2
  Relational49/1 -> Delay131/1
  Mux47/1 -> AddSub51/1, Delay174/1
  Delay160/1 -> Mux44/1
  Delay146/1 -> Delay149/1, Relational54/1
  Mux44/1 -> AddSub48/1, Delay164/1
  AddSub47/1 -> Mux44/3
  Mux50/1 -> AddSub52/1, Delay144/1
  Delay157/1 -> Mux55/2
  Delay149/1 -> Delay152/1, Relational55/1
  Mux52/1 -> AddSub55/1, Delay151/1
  Mux41/1 -> Delay129/1, AddSub60/1
  Delay172/1 -> Relational50/1, Delay175/1
  Delay153/1 -> Mux54/1
  Delay156/1 -> Mux55/1
  AddSub49/1 -> Mux46/3
  Delay155/1 -> Relational58/1, Delay132/1
  Relational44/1 -> Delay160/1
  Delay169/1 -> Delay172/1, Relational48/1
  Delay151/1 -> Mux53/2
  Delay163/1 -> Mux45/1
  Relational48/1 -> Delay173/1
  Delay171/1 -> Mux47/2
  Relational54/1 -> Delay150/1
  Delay124/1 -> Mux42/1
  Delay159/1 -> Relational44/1, Delay162/1
  logi_b20/1 -> Relational43/2, Relational49/2
  Delay150/1 -> Mux53/1
  Delay131/1 -> Mux13/1
  Delay174/1 -> Mux48/2
  AddSub57/1 -> Mux55/3
  Delay148/1 -> Mux52/2
  AddSub54/1 -> Mux52/3
  Mux55/1 -> AddSub59/1, Delay134/1
  Delay119/1 -> Relational42/1, Delay126/1
  Delay136/1 -> Mux56/1
  Delay158/1 -> Mux43/2
  AddSub77/1 -> Mux86/3
  Mux75/1 -> AddSub111/1, Delay189/1
  Delay271/1 -> Relational72/1, Delay274/1
  AddSub97/1 -> Mux106/3
  AddSub65/1 -> Mux63/3
  AddSub95/1 -> Mux92/3
  Relational80/1 -> Delay298/1
  Delay268/1 -> Relational60/1, Delay185/1
  Relational65/1 -> Delay323/1
  logi_b45/1 -> Relational89/2, Relational88/2
  Delay298/1 -> Mux81/1
  Delay237/1 -> Relational91/1, Delay241/1
  Delay220/1 -> Mux99/1
  Relational96/1 -> Delay207/1
  Relational62/1 -> Delay182/1
  Delay200/1 -> Mux89/2
  Delay272/1 -> Mux70/1
  Relational89/1 -> Delay199/1
  Delay206/1 -> Delay215/1, Relational96/1
  AddSub79/1 -> Mux76/3
  Delay203/1 -> Mux58/1
  Mux91/1 -> AddSub95/1, Delay243/1
  AddSub100/1 -> Mux99/3
  Delay307/1 -> Relational84/1, Delay310/1
  Mux78/1 -> AddSub82/1, Delay178/1
  AddSub74/1 -> Mux72/3
  Delay239/1 -> Mux91/1
  Mux69/1 -> AddSub72/1, Delay273/1
  Delay243/1 -> Mux92/2
  AddSub68/1 -> Mux66/3
  Relational90/1 -> Delay202/1
  AddSub91/1 -> Mux98/3
  Mux107/1 -> AddSub110/1, Delay267/1
  logi_b47/1 -> Relational91/2, Relational99/2
  Delay304/1 -> Delay307/1, Relational83/1
  logi_b48/1 -> Relational92/2, Relational100/2
  Delay194/1 -> Mux77/1
  AddSub90/1 -> Mux61/3
  Delay262/1 -> Relational110/1, Delay265/1
  Relational79/1 -> Delay295/1
  Delay218/1 -> Mux98/2
  Delay322/1 -> Delay325/1, Relational66/1
  AddSub111/1 -> Mux109/3
  AddSub76/1 -> Mux74/3
  Delay285/1 -> Mux74/1
  Delay294/1 -> Relational79/1, Delay297/1
  Delay202/1 -> Mux90/1
  Delay329/1 -> Mux78/1
  logi_b30/1 -> Relational73/2, Relational97/2
  AddSub109/1 -> Mux58/3
  AddSub70/1 -> Mux77/3
  Delay240/1 -> Mux91/2
  Delay236/1 -> Mux90/2
  Relational60/1 -> Delay183/1
  Delay205/1 -> Mux77/2
  Delay204/1 -> Mux58/2
  Delay191/1 -> Mux88/1
  Mux63/1 -> AddSub66/1, Delay316/1
  Delay328/1 -> Relational69/1, Delay331/1
  Delay266/1 -> Mux108/1
  Delay257/1 -> Mux97/1
  Delay326/1 -> Mux67/1
  Delay331/1 -> Relational85/1, Delay193/1
  Delay287/1 -> Relational59/1, Delay291/1
  AddSub88/1 -> Mux87/3
  Delay309/1 -> Mux84/2
  Relational92/1 -> Delay242/1
  Delay217/1 -> Mux98/1
  Mux70/1 -> AddSub73/1, Delay276/1
  Delay190/1 -> Relational88/1, Delay206/1
  Mux67/1 -> AddSub80/1, Delay330/1
  Delay193/1 -> Relational89/1, Delay201/1
  Delay324/1 -> Mux66/2
  Delay178/1 -> Mux79/2
  Delay177/1 -> Mux79/1
  Mux59/1 -> AddSub62/1, Delay293/1
  Mux64/1 -> AddSub67/1, Delay319/1
  Delay275/1 -> Mux71/1
  Delay219/1 -> Relational100/1, Delay222/1
  logi_b36/1 -> Relational61/2, Relational60/2
  Delay267/1 -> Mux108/2
  Relational85/1 -> Delay195/1
  Delay185/1 -> Delay294/1, Relational68/1
  AddSub92/1 -> Mux89/3
  Mux108/1 -> AddSub79/1, Delay290/1
  Relational88/1 -> Delay203/1
  Mux109/1 -> Delay180/1, AddSub64/1
  Relational91/1 -> Delay239/1
  Relational66/1 -> Delay326/1
  Delay278/1 -> Delay281/1, Relational75/1
  Mux88/1 -> Delay204/1, AddSub109/1
  Mux86/1 -> AddSub87/1, Delay258/1
  Delay310/1 -> Relational87/1, Delay190/1
  Relational99/1 -> Delay217/1
  AddSub63/1 -> Mux80/3
  logi_b40/1 -> Relational65/2, Relational81/2
  AddSub89/1 -> Mux88/3
  Mux82/1 -> AddSub84/1, Delay306/1
  Delay196/1 -> Mux87/2
  Relational69/1 -> Delay177/1
  Mux56/1 -> Delay270/1, AddSub71/1
  Relational64/1 -> Delay318/1
  Mux83/1 -> AddSub85/1, Delay309/1
  Relational75/1 -> Delay282/1
  logi_b39/1 -> Relational64/2, Relational80/2
  Mux62/1 -> AddSub65/1, Delay313/1
  logi_b41/1 -> Relational66/2, Relational82/2
  Delay288/1 -> Mux75/1
  AddSub85/1 -> Mux84/3
  Delay241/1 -> Relational92/1, Delay244/1
  Delay281/1 -> Delay284/1, Relational76/1
  Delay215/1 -> Relational99/1, Delay219/1
  Delay207/1 -> Mux61/1
  Mux87/1 -> Delay200/1, AddSub92/1
  Delay265/1 -> Relational70/1, Delay268/1
  Delay264/1 -> Mux107/2
  Relational61/1 -> Delay179/1
  Delay301/1 -> Delay304/1, Relational82/1
  AddSub72/1 -> Mux70/3
  AddSub80/1 -> Mux78/3
  Delay189/1 -> Mux109/2
  Relational100/1 -> Delay220/1
  AddSub61/1 -> Mux68/3
  AddSub112/1 -> Mux59/3
  Delay199/1 -> Mux89/1
  Delay317/1 -> Relational64/1, Delay320/1
  Delay289/1 -> Mux75/2
  Mux66/1 -> AddSub69/1, Delay327/1
  Delay192/1 -> Mux88/2
  logi_b35/1 -> Relational59/2, Relational70/2
  Delay291/1 -> Relational61/1, Delay181/1
  AddSub71/1 -> Mux69/3
  Mux84/1 -> AddSub86/1, Delay312/1
  Delay259/1 -> Delay262/1, Relational109/1
  Delay302/1 -> Mux82/1
  AddSub64/1 -> Mux62/3
  Delay221/1 -> Mux99/2
  Delay269/1 -> Mux76/1
  Delay305/1 -> Mux83/1
  Mux77/1 -> AddSub77/1, Delay238/1
  Relational68/1 -> Delay186/1
  Delay321/1 -> Mux68/1
  Delay263/1 -> Mux107/1
  AddSub93/1 -> Mux90/3
  AddSub81/1 -> Mux81/3
  Delay315/1 -> Mux64/1
  Delay184/1 -> Mux59/2
  Delay311/1 -> Mux85/1
  Relational81/1 -> Delay302/1
  Delay318/1 -> Mux65/1
  Delay316/1 -> Mux64/2
  Relational70/1 -> Delay269/1
  Mux79/1 -> AddSub88/1, Delay196/1
  logi_b28/1 -> Relational71/2, Relational77/2
  logi_b46/1 -> Relational90/2, Relational96/2
  Delay183/1 -> Mux59/1
  Mux68/1 -> AddSub70/1, Delay205/1
  Delay300/1 -> Delay301/1, Relational81/1
  logi_b42/1 -> Relational67/2, Relational83/2
  Relational107/1 -> Delay257/1
  AddSub94/1 -> Mux91/3
  Delay276/1 -> Mux71/2
  Delay274/1 -> Relational73/1, Delay277/1
  Delay249/1 -> Delay256/1, Relational107/1
  AddSub110/1 -> Mux108/3
  Delay290/1 -> Mux76/2
  Relational73/1 -> Delay275/1
  Mux74/1 -> AddSub78/1, Delay289/1
  Delay258/1 -> Mux97/2
  AddSub87/1 -> Mux97/3
  Mux97/1 -> AddSub97/1, Delay261/1
  Delay312/1 -> Mux85/2
  Delay216/1 -> Relational97/1, Delay249/1
  Delay135/1 -> Delay271/1, Relational71/1
  AddSub73/1 -> Mux71/3
  Delay277/1 -> Delay278/1, Relational74/1
  Relational78/1 -> Delay288/1
  logi_b44/1 -> Relational85/2, Relational87/2
  Delay260/1 -> Mux106/1
  Mux61/1 -> AddSub91/1, Delay218/1
  logi_b32/1 -> Relational75/2, Relational108/2
  Delay214/1 -> Mux61/2
  Delay238/1 -> Mux86/2
  Relational110/1 -> Delay266/1
  Relational84/1 -> Delay311/1
  logi_b43/1 -> Relational69/2, Relational84/2
  AddSub84/1 -> Mux83/3
  Mux81/1 -> AddSub83/1, Delay303/1
  Mux65/1 -> AddSub68/1, Delay324/1
  Delay319/1 -> Mux65/2
  Delay297/1 -> Relational80/1, Delay300/1
  AddSub82/1 -> Mux79/3
  Relational67/1 -> Delay329/1
  Delay299/1 -> Mux81/2
  Relational83/1 -> Delay308/1
  Relational72/1 -> Delay272/1
  Delay292/1 -> Mux69/1
  Delay282/1 -> Mux73/1
  Mux57/1 -> Delay176/1, AddSub61/1
  Delay283/1 -> Mux73/2
  Relational77/1 -> Delay321/1
  Mux89/1 -> AddSub93/1, Delay236/1
  Delay132/1 -> Delay187/1, Relational77/1
  Delay242/1 -> Mux92/1
  Delay303/1 -> Mux82/2
  Mux58/1 -> AddSub90/1, Delay214/1
  Delay284/1 -> Relational78/1, Delay287/1
  Mux98/1 -> AddSub100/1, Delay221/1
  Relational87/1 -> Delay191/1
  Delay201/1 -> Delay237/1, Relational90/1
  Delay306/1 -> Mux83/2
  Mux90/1 -> AddSub94/1, Delay240/1
  Mux76/1 -> Delay184/1, AddSub112/1
  Mux71/1 -> AddSub74/1, Delay280/1
  AddSub78/1 -> Mux75/3
  Delay286/1 -> Mux74/2
  Delay180/1 -> Mux62/2
  Delay296/1 -> Mux80/2
  Delay293/1 -> Mux60/2
  AddSub69/1 -> Mux67/3
  AddSub62/1 -> Mux60/3
  Delay295/1 -> Mux80/1
  Mux60/1 -> AddSub63/1, Delay296/1
  Delay182/1 -> Mux63/1
  AddSub83/1 -> Mux82/3
  Relational59/1 -> Delay188/1
  Relational63/1 -> Delay315/1
  Delay181/1 -> Delay314/1, Relational62/1
  Delay320/1 -> Delay322/1, Relational65/1
  Delay325/1 -> Delay328/1, Relational67/1
  Delay323/1 -> Mux66/1
  Mux80/1 -> AddSub81/1, Delay299/1
  AddSub66/1 -> Mux64/3
  Delay327/1 -> Mux67/2
  logi_b38/1 -> Relational63/2, Relational79/2
  Relational82/1 -> Delay305/1
  Delay179/1 -> Mux62/1
  Delay314/1 -> Relational63/1, Delay317/1
  logi_b37/1 -> Relational62/2, Relational68/2
  AddSub67/1 -> Mux65/3
  Delay186/1 -> Mux60/1
  Delay308/1 -> Mux84/1
  Delay330/1 -> Mux78/2
  AddSub86/1 -> Mux85/3
  Mux85/1 -> AddSub89/1, Delay192/1
  Relational71/1 -> Delay292/1
  Delay227/1 -> Mux86/1
  Mux73/1 -> AddSub76/1, Delay286/1
  logi_b34/1 -> Relational78/2, Relational110/2
  Delay280/1 -> Mux72/2
  Mux72/1 -> AddSub75/1, Delay283/1
  Delay273/1 -> Mux70/2
  Relational109/1 -> Delay263/1
  logi_b29/1 -> Relational72/2, Relational86/2
  Delay261/1 -> Mux106/2
  Relational76/1 -> Delay285/1
  Delay313/1 -> Mux63/2
  logi_b33/1 -> Relational76/2, Relational109/2
  Relational108/1 -> Delay260/1
  Delay195/1 -> Mux87/1
  Relational86/1 -> Delay194/1
  Relational97/1 -> Delay227/1
  Mux106/1 -> AddSub108/1, Delay264/1
  Delay176/1 -> Mux68/2
  AddSub75/1 -> Mux73/3
  Delay256/1 -> Delay259/1, Relational108/1
  logi_b31/1 -> Relational74/2, Relational107/2
  Delay270/1 -> Mux69/2
  AddSub108/1 -> Mux107/3
  Delay188/1 -> Mux109/1
  Delay187/1 -> Relational86/1, Delay216/1
  Delay279/1 -> Mux72/1
  Relational74/1 -> Delay279/1
  Scaling/1 -> Gateway Out/1
  Slice2/1 -> AddSub20/2
  AddSub201/1 -> Mux100/3
  Mux114/1 -> AddSub118/1, Delay591/1
  logi_b56/1 -> Relational129/2, Relational185/2
  logi_b84/1 -> Relational162/2, Relational175/2
  AddSub161/1 -> Mux172/3
  Delay335/1 -> Mux143/1
  logi_b83/1 -> Relational183/2, Relational106/2
  AddSub99/1 -> Mux117/3
  Relational159/1 -> Delay367/1
  Delay453/1 -> Mux100/2
  AddSub122/1 -> Mux120/3
  Relational164/1 -> Delay397/1
  AddSub193/1 -> Mux192/3
  Delay563/1 -> Mux132/1
  Delay224/1 -> Mux112/1
  Relational118/1 -> Delay229/1
  Delay440/1 -> Mux196/2
  AddSub101/1 -> Mux105/3
  Delay466/1 -> Mux173/2
  Delay376/1 -> Mux145/2
  Relational131/1 -> Delay548/1
  Delay235/1 -> Mux194/1
  Relational117/1 -> Delay596/1
  logi_b66/1 -> Relational120/2, Relational137/2
  Mux161/1 -> AddSub161/1, Delay451/1
  AddSub119/1 -> Mux116/3
  Mux117/1 -> AddSub120/1, Delay338/1
  AddSub102/1 -> Mux200/3
  Delay347/1 -> Mux110/2
  Delay254/1 -> Mux149/1
  logi_b60/1 -> Relational112/2, Relational118/2
  Delay464/1 -> Relational177/1, Delay467/1
  AddSub152/1 -> Mux148/3
  Relational102/1 -> Delay448/1
  Delay226/1 -> Mux104/2
  Delay233/1 -> Mux137/1
  Delay424/1 -> Relational202/1, Delay428/1
  Delay351/1 -> Mux151/2
  Delay549/1 -> Mux126/2
  AddSub128/1 -> Mux139/3
  Relational127/1 -> Delay538/1
  Mux181/1 -> AddSub186/1, Delay391/1
  AddSub190/1 -> Mux189/3
  Relational183/1 -> Delay482/1
  logi_b94/1 -> Relational195/2, Relational194/2
  logi_b95/1 -> Relational197/2, Relational200/2
  Delay368/1 -> Mux156/2
  Relational192/1 -> Delay409/1
  Delay469/1 -> Mux174/2
  Mux136/1 -> AddSub142/1, Delay248/1
  Delay373/1 -> Mux144/2
  AddSub169/1 -> Mux167/3
  Delay364/1 -> Mux155/1
  Delay359/1 -> Delay363/1, Relational158/1
  Mux124/1 -> AddSub127/1, Delay545/1
  Delay421/1 -> Mux163/1
  Delay411/1 -> Mux191/2
  AddSub137/1 -> Mux136/3
  Relational190/1 -> Delay508/1
  Delay491/1 -> Mux184/2
  logi_b89/1 -> Relational169/2, Relational187/2
  Mux186/1 -> AddSub188/1, Delay502/1
  logi_b62/1 -> Relational114/2, Relational133/2
  Delay493/1 -> Mux185/1
  Delay520/1 -> Delay523/1, Relational170/1
  AddSub151/1 -> Mux147/3
  Delay443/1 -> Mux197/2
  AddSub184/1 -> Mux181/3
  Delay427/1 -> Mux199/2
  Delay255/1 -> Mux149/2
  Relational114/1 -> Delay585/1
  logi_b79/1 -> Relational178/2, Relational201/2
  logi_b64/1 -> Relational116/2, Relational135/2
  AddSub155/1 -> Mux153/3
  Delay494/1 -> Mux185/2
  Delay379/1 -> Mux146/1
  AddSub164/1 -> Mux162/3
  AddSub171/1 -> Mux169/3
  AddSub166/1 -> Mux164/3
  Mux163/1 -> AddSub196/1, Delay427/1
  Relational157/1 -> Delay361/1
  Mux125/1 -> AddSub129/1, Delay549/1
  Delay213/1 -> Mux111/2
  Relational126/1 -> Delay534/1
  Constant7/1 -> AddSub12/2, AddSub45/2, AddSub64/2, AddSub92/2, AddSub121/2, AddSub114/2, AddSub145/2, AddSub166/2, AddSub197/2, AddSub236/2, AddSub298/2, AddSub297/2, AddSub296/2, AddSub295/2, AddSub290/2, AddSub284/2, AddSub282/2, AddSub269/2, AddSub268/2, AddSub267/2, AddSub266/2, AddSub265/2, AddSub264/2, AddSub210/2, AddSub279/2, AddSub277/2, AddSub276/2, AddSub275/2, AddSub274/2, AddSub273/2, AddSub272/2, AddSub257/2, AddSub252/2, AddSub250/2, AddSub249/2, AddSub138/2, AddSub200/2, AddSub199/2, AddSub198/2, AddSub192/2, AddSub186/2, AddSub184/2, AddSub171/2, AddSub170/2, AddSub169/2, AddSub168/2, AddSub167/2, AddSub107/2, AddSub181/2, AddSub179/2, AddSub178/2, AddSub177/2, AddSub176/2, AddSub175/2, AddSub174/2, AddSub159/2, AddSub154/2, AddSub152/2, AddSub151/2, AddSub149/2, AddSub148/2, AddSub147/2, AddSub146/2, AddSub141/2, AddSub133/2, AddSub131/2, AddSub119/2, AddSub118/2, AddSub117/2, AddSub116/2, AddSub115/2, AddSub183/2, AddSub129/2, AddSub127/2, AddSub126/2, AddSub125/2, AddSub124/2, AddSub123/2, AddSub122/2, AddSub39/2, AddSub95/2, AddSub94/2, AddSub93/2, AddSub88/2, AddSub82/2, AddSub80/2, AddSub69/2, AddSub68/2, AddSub67/2, AddSub66/2, AddSub65/2, AddSub111/2, AddSub78/2, AddSub76/2, AddSub75/2, AddSub74/2, AddSub73/2, AddSub72/2, AddSub71/2, AddSub58/2, AddSub53/2, AddSub51/2, AddSub50/2, AddSub49/2, AddSub48/2, AddSub47/2, AddSub46/2, AddSub41/2, AddSub34/2, AddSub32/2, AddSub17/2, AddSub16/2, AddSub15/2, AddSub14/2, AddSub13/2, AddSub8/2, AddSub30/2, AddSub29/2, AddSub28/2, AddSub27/2, AddSub26/2, AddSub25/2, AddSub24/2, AddSub23/2, Mux20/3
  Delay406/1 -> Mux192/1
  Delay434/1 -> Mux161/2
  Delay558/1 -> Mux105/2
  Delay253/1 -> Mux140/2
  Mux158/1 -> Delay389/1, AddSub163/1
  Delay410/1 -> Mux191/1
  Mux100/1 -> AddSub103/1, Delay456/1
  Delay471/1 -> Delay475/1, Relational180/1
  Delay576/1 -> Relational142/1, Delay246/1
  Delay554/1 -> Mux119/2
  Relational187/1 -> Delay498/1
  Delay407/1 -> Mux192/2
  Delay577/1 -> Relational130/1, Delay230/1
  Delay225/1 -> Mux104/1
  Mux171/1 -> AddSub175/1, Delay466/1
  Delay588/1 -> Mux117/1
  Mux177/1 -> AddSub181/1, Delay483/1
  Relational201/1 -> Delay433/1
  Mux123/1 -> AddSub126/1, Delay542/1
  logi_b85/1 -> Relational165/2, Relational164/2
  Delay403/1 -> Mux103/2
  Delay417/1 -> Mux159/1
  Relational95/1 -> Delay557/1
  Delay229/1 -> Mux105/1
  AddSub162/1 -> Mux96/3
  logi_b59/1 -> Relational111/2, Relational105/2
  Relational188/1 -> Delay501/1
  AddSub114/1 -> Mux111/3
  Delay523/1 -> Delay526/1, Relational171/1
  AddSub120/1 -> Mux128/3
  AddSub117/1 -> Mux114/3
  Delay365/1 -> Mux155/2
  Mux105/1 -> AddSub105/1, Delay561/1
  Delay445/1 -> Delay447/1, Relational102/1
  Mux115/1 -> AddSub119/1, Delay594/1
  Relational148/1 -> Delay379/1
  Delay348/1 -> Relational154/1, Delay352/1
  Delay509/1 -> Mux189/2
  Relational195/1 -> Delay412/1
  Delay536/1 -> Delay537/1, Relational127/1
  Delay418/1 -> Mux159/2
  AddSub199/1 -> Mux196/3
  Mux154/1 -> AddSub157/1, Delay365/1
  Delay234/1 -> Mux137/2
  Relational153/1 -> Delay254/1
  Mux38/1 -> Delay554/1, AddSub121/1
  Delay429/1 -> Mux161/1
  AddSub158/1 -> Mux156/3
  Delay370/1 -> Relational146/1, Delay374/1
  Delay535/1 -> Mux122/2
  Delay209/1 -> Mux117/2
  Relational143/1 -> Delay336/1
  Delay528/1 -> Relational125/1, Delay533/1
  Delay552/1 -> Delay555/1, Relational121/1
  Delay349/1 -> Relational152/1, Delay382/1
  Delay470/1 -> Delay471/1, Relational179/1
  Delay580/1 -> Mux112/2
  Delay419/1 -> Mux180/2
  Delay486/1 -> Relational165/1, Delay395/1
  Delay366/1 -> Relational161/1, Delay341/1
  Mux160/1 -> AddSub164/1, Delay488/1
  Mux190/1 -> AddSub191/1, Delay449/1
  Relational186/1 -> Delay493/1
  AddSub185/1 -> Mux185/3
  Mux200/1 -> AddSub140/1, Delay232/1
  Delay385/1 -> Relational153/1, Delay388/1
  AddSub187/1 -> Mux186/3
  Delay513/1 -> Mux166/2
  Delay504/1 -> Mux188/1
  Delay390/1 -> Mux182/1
  logi_b65/1 -> Relational117/2, Relational136/2
  Relational202/1 -> Delay426/1
  Delay468/1 -> Mux174/1
  Relational168/1 -> Delay515/1
  Delay409/1 -> Mux180/1
  AddSub174/1 -> Mux171/3
  AddSub125/1 -> Mux123/3
  Mux129/1 -> AddSub133/1, Delay211/1
  Delay518/1 -> Delay520/1, Relational169/1
  Mux194/1 -> Delay213/1, AddSub114/1
  Mux101/1 -> AddSub106/1, Delay459/1
  Relational140/1 -> Delay252/1
  Delay527/1 -> Mux181/1
  Delay598/1 -> Relational140/1, Delay250/1
  AddSub156/1 -> Mux154/3
  Mux102/1 -> AddSub182/1, Delay485/1
  Relational177/1 -> Delay465/1
  Relational184/1 -> Delay490/1
  AddSub179/1 -> Mux177/3
  Delay481/1 -> Relational162/1, Delay486/1
  Delay555/1 -> Delay528/1, Relational124/1
  Delay381/1 -> Delay385/1, Relational150/1
  Mux172/1 -> AddSub172/1, Delay484/1
  Delay533/1 -> Relational126/1, Delay536/1
  Relational120/1 -> Delay210/1
  Mux183/1 -> AddSub130/1, Delay550/1
  AddSub191/1 -> Mux198/3
  Mux159/1 -> AddSub195/1, Delay423/1
  Mux149/1 -> AddSub159/1, Delay346/1
  Delay568/1 -> Mux133/1
  Delay566/1 -> Mux95/2
  Delay246/1 -> Relational143/1, Delay339/1
  Delay505/1 -> Mux188/2
  logi_b93/1 -> Relational191/2, Relational193/2
  Delay228/1 -> Delay559/1, Relational118/1
  Mux120/1 -> AddSub123/1, Delay532/1
  Relational178/1 -> Delay468/1
  Delay382/1 -> Delay393/1, Relational163/1
  Delay562/1 -> Relational133/1, Delay565/1
  Delay448/1 -> Mux198/1
  Delay355/1 -> Delay356/1, Relational156/1
  Delay371/1 -> Mux139/2
  AddSub196/1 -> Mux199/3
  Mux116/1 -> AddSub131/1, Delay597/1
  Delay451/1 -> Mux172/2
  Relational104/1 -> Delay455/1
  Delay567/1 -> Delay570/1, Relational135/1
  Relational191/1 -> Delay410/1
  Delay346/1 -> Mux157/2
  Delay245/1 -> Mux194/2
  Delay575/1 -> Mux135/2
  Relational175/1 -> Delay461/1
  Delay551/1 -> Relational111/1, Delay223/1
  Delay425/1 -> Relational201/1, Delay445/1
  Mux157/1 -> Delay463/1, AddSub174/1
  Delay455/1 -> Mux101/1
  AddSub175/1 -> Mux173/3
  Delay447/1 -> Delay450/1, Relational103/1
  Delay353/1 -> Mux152/1
  Delay502/1 -> Mux187/2
  Delay537/1 -> Delay540/1, Relational128/1
  logi_b77/1 -> Relational176/2, Relational182/2
  AddSub113/1 -> Mux160/3
  logi_b87/1 -> Relational167/2, Relational184/2
  Delay510/1 -> Mux165/2
  AddSub186/1 -> Mux182/3
  Delay404/1 -> Mux150/1
  Delay482/1 -> Mux178/1
  Delay503/1 -> Relational190/1, Delay507/1
  AddSub132/1 -> Mux132/3
  Relational149/1 -> Delay383/1
  Mux128/1 -> AddSub128/1, Delay371/1
  logi_b63/1 -> Relational115/2, Relational134/2
  logi_b52/1 -> Relational125/2, Relational141/2
  Delay387/1 -> Mux148/2
  AddSub176/1 -> Mux174/3
  AddSub146/1 -> Mux143/3
  AddSub170/1 -> Mux168/3
  Delay472/1 -> Mux175/1
  Delay352/1 -> Relational155/1, Delay355/1
  Delay538/1 -> Mux123/1
  Relational160/1 -> Delay345/1
  Delay250/1 -> Relational144/1, Delay334/1
  AddSub159/1 -> Mux157/3
  AddSub177/1 -> Mux175/3
  Relational198/1 -> Delay438/1
  Delay487/1 -> Mux171/1
  Delay476/1 -> Mux176/1
  Delay211/1 -> Mux130/2
  AddSub153/1 -> Mux152/3
  Delay595/1 -> Relational120/1, Delay598/1
  Delay452/1 -> Mux100/1
  Delay446/1 -> Mux172/1
  Relational200/1 -> Delay421/1
  Delay449/1 -> Mux198/2
  Relational166/1 -> Delay396/1
  Delay572/1 -> Mux134/2
  Delay454/1 -> Relational106/1, Delay457/1
  Delay383/1 -> Mux147/1
  Mux176/1 -> AddSub179/1, Delay480/1
  logi_b55/1 -> Relational128/2, Relational174/2
  Mux143/1 -> AddSub147/1, Delay373/1
  Mux169/1 -> AddSub184/1, Delay529/1
  Delay336/1 -> Mux96/1
  Delay507/1 -> Relational193/1, Delay405/1
  Relational197/1 -> Delay416/1
  Mux148/1 -> AddSub154/1, Delay255/1
  AddSub194/1 -> Mux104/3
  Mux142/1 -> AddSub146/1, Delay369/1
  logi_b61/1 -> Relational113/2, Relational132/2
  Delay460/1 -> Relational164/1, Delay399/1
  Relational125/1 -> Delay531/1
  Relational165/1 -> Delay392/1
  Delay475/1 -> Delay478/1, Relational181/1
  Delay483/1 -> Mux178/2
  Relational105/1 -> Delay225/1
  Delay232/1 -> Mux138/2
  Relational122/1 -> Delay506/1
  Delay539/1 -> Mux123/2
  AddSub148/1 -> Mux145/3
  Mux141/1 -> Delay337/1, AddSub162/1
  AddSub141/1 -> Mux140/3
  Delay584/1 -> Relational114/1, Delay587/1
  Mux103/1 -> Delay394/1, AddSub166/1
  AddSub150/1 -> Mux161/3
  Mux189/1 -> AddSub193/1, Delay407/1
  logi_b73/1 -> Relational149/2, Relational157/2
  Relational163/1 -> Delay404/1
  Delay413/1 -> Mux150/2
  Delay530/1 -> Relational191/1, Delay408/1
  Delay360/1 -> Mux139/1
  logi_b91/1 -> Relational171/2, Relational189/2
  Mux193/1 -> AddSub198/1, Delay435/1
  logi_b82/1 -> Relational181/2, Relational104/2
  Mux180/1 -> AddSub180/1, Delay437/1
  Delay574/1 -> Mux135/1
  Mux185/1 -> AddSub187/1, Delay499/1
  Delay345/1 -> Mux157/1
  Delay393/1 -> Delay422/1, Relational174/1
  AddSub167/1 -> Mux165/3
  Delay531/1 -> Mux121/1
  logi_b90/1 -> Relational170/2, Relational188/2
  Mux188/1 -> AddSub190/1, Delay509/1
  AddSub178/1 -> Mux176/3
  Delay508/1 -> Mux189/1
  Delay212/1 -> Mux111/1
  Delay426/1 -> Mux199/1
  Delay581/1 -> Relational113/1, Delay584/1
  Relational142/1 -> Delay247/1
  Delay412/1 -> Mux193/1
  logi_b54/1 -> Relational127/2, Relational163/2
  Mux111/1 -> AddSub115/1, Delay580/1
  Mux96/1 -> AddSub143/1, Delay347/1
  logi_b50/1 -> Relational121/2, Relational95/2
  Delay251/1 -> Mux128/1
  Relational103/1 -> Delay452/1
  Delay431/1 -> Mux200/2
  AddSub145/1 -> Mux142/3
  Delay392/1 -> Mux164/1
  logi_b58/1 -> Relational98/2, Relational122/2
  Relational111/1 -> Delay212/1
  Mux195/1 -> AddSub199/1, Delay440/1
  Delay405/1 -> Relational194/1, Delay420/1
  AddSub142/1 -> Mux141/3
  Delay565/1 -> Delay567/1, Relational134/1
  Delay369/1 -> Mux143/2
  Delay433/1 -> Mux190/1
  Delay501/1 -> Mux187/1
  Relational139/1 -> Delay233/1
  Mux167/1 -> AddSub170/1, Delay522/1
  Delay465/1 -> Mux173/1
  Delay231/1 -> Mux138/1
  Delay479/1 -> Mux177/1
  AddSub138/1 -> Mux137/3
  Relational156/1 -> Delay357/1
  AddSub157/1 -> Mux155/3
  Delay540/1 -> Delay543/1, Relational129/1
  AddSub143/1 -> Mux110/3
  Delay372/1 -> Mux144/1
  Delay450/1 -> Delay454/1, Relational104/1
  Delay252/1 -> Mux140/1
  Delay556/1 -> Mux120/1
  Delay357/1 -> Mux153/1
  Delay485/1 -> Mux179/2
  Mux198/1 -> AddSub201/1, Delay453/1
  Delay546/1 -> Relational98/1, Delay551/1
  Delay338/1 -> Mux128/2
  logi_b98/1 -> Relational139/2, Relational138/2
  Relational180/1 -> Delay476/1
  Delay344/1 -> Delay464/1, Relational176/1
  Delay400/1 -> Mux162/1
  Delay395/1 -> Delay511/1, Relational166/1
  Delay514/1 -> Relational168/1, Delay518/1
  Mux145/1 -> AddSub149/1, Delay380/1
  Mux196/1 -> AddSub200/1, Delay443/1
  Mux155/1 -> AddSub158/1, Delay368/1
  AddSub103/1 -> Mux101/3
  Delay230/1 -> Relational141/1, Delay349/1
  Delay399/1 -> Delay489/1, Relational172/1
  Mux152/1 -> AddSub155/1, Delay358/1
  Delay561/1 -> Mux131/2
  Delay548/1 -> Mux126/1
  AddSub183/1 -> Mux194/3
  Delay401/1 -> Relational192/1, Delay425/1
  Delay499/1 -> Mux186/2
  Delay545/1 -> Mux125/2
  Delay474/1 -> Mux175/2
  Delay332/1 -> Mux142/1
  Relational182/1 -> Delay519/1
  Delay461/1 -> Mux179/1
  AddSub129/1 -> Mux126/3
  Delay495/1 -> Relational105/1, Delay228/1
  Delay532/1 -> Mux121/2
  Mux119/1 -> AddSub122/1, Delay517/1
  AddSub115/1 -> Mux112/3
  Delay543/1 -> Relational131/1, Delay546/1
  Delay498/1 -> Mux186/1
  Delay389/1 -> Mux170/2
  Relational124/1 -> Delay556/1
  Mux110/1 -> AddSub144/1, Delay351/1
  Delay361/1 -> Mux154/1
  AddSub126/1 -> Mux124/3
  Mux179/1 -> Delay398/1, AddSub113/1
  Delay416/1 -> Mux195/1
  Delay463/1 -> Mux171/2
  Delay343/1 -> Mux158/2
  Delay596/1 -> Mux129/1
  Mux147/1 -> AddSub152/1, Delay387/1
  Delay490/1 -> Mux184/1
  Delay396/1 -> Mux165/1
  Mux165/1 -> AddSub168/1, Delay513/1
  AddSub168/1 -> Mux166/3
  Mux199/1 -> AddSub102/1, Delay431/1
  Mux122/1 -> AddSub125/1, Delay539/1
  AddSub198/1 -> Mux195/3
  Delay521/1 -> Mux168/1
  AddSub135/1 -> Mux134/3
  Delay560/1 -> Mux131/1
  logi_b72/1 -> Relational148/2, Relational156/2
  logi_b97/1 -> Relational199/2, Relational101/2
  Relational158/1 -> Delay364/1
  Relational167/1 -> Delay512/1
  Delay597/1 -> Mux129/2
  Delay582/1 -> Mux113/1
  Relational179/1 -> Delay472/1
  AddSub192/1 -> Mux191/3
  Delay541/1 -> Mux124/1
  Delay435/1 -> Mux195/2
  Delay437/1 -> Mux190/2
  AddSub130/1 -> Mux127/3
  Delay374/1 -> Relational147/1, Delay377/1
  Delay512/1 -> Mux166/1
  AddSub105/1 -> Mux131/3
  Mux39/1 -> Delay566/1, AddSub98/1
  Delay398/1 -> Mux160/2
  Relational196/1 -> Delay473/1
  Relational155/1 -> Delay353/1
  logi_b96/1 -> Relational198/2, Relational202/2
  Mux178/1 -> AddSub107/1, Delay403/1
  AddSub182/1 -> Mux179/3
  Mux150/1 -> AddSub150/1, Delay434/1
  Delay342/1 -> Mux158/1
  Relational170/1 -> Delay524/1
  Delay578/1 -> Mux136/1
  Delay534/1 -> Mux122/1
  Delay571/1 -> Mux134/1
  Relational132/1 -> Delay560/1
  Relational181/1 -> Delay479/1
  Relational169/1 -> Delay521/1
  Relational152/1 -> Delay360/1
  Delay339/1 -> Delay348/1, Relational151/1
  AddSub173/1 -> Mux180/3
  Mux121/1 -> AddSub124/1, Delay535/1
  Relational135/1 -> Delay571/1
  Relational134/1 -> Delay568/1
  AddSub160/1 -> Mux158/3
  Mux164/1 -> AddSub167/1, Delay510/1
  AddSub197/1 -> Mux193/3
  Relational98/1 -> Delay235/1
  Mux139/1 -> AddSub139/1, Delay413/1
  Delay579/1 -> Mux136/2
  Relational194/1 -> Delay417/1
  Delay524/1 -> Mux169/1
  Delay408/1 -> Relational195/1, Delay415/1
  logi_b53/1 -> Relational126/2, Relational152/2
  Delay516/1 -> Mux167/2
  logi_b81/1 -> Relational180/2, Relational103/2
  AddSub104/1 -> Mux159/3
  Delay391/1 -> Mux182/2
  Delay356/1 -> Delay359/1, Relational157/1
  Delay593/1 -> Mux116/1
  Delay564/1 -> Mux132/2
  Relational101/1 -> Delay430/1
  Relational128/1 -> Delay541/1
  Delay506/1 -> Mux127/1
  Delay456/1 -> Mux101/2
  logi_b57/1 -> Relational131/2, Relational196/2
  logi_b88/1 -> Relational168/2, Relational186/2
  Delay438/1 -> Mux196/1
  Delay384/1 -> Mux147/2
  Delay340/1 -> Mux110/1
  Relational161/1 -> Delay342/1
  Mux134/1 -> AddSub136/1, Delay575/1
  Mux175/1 -> AddSub178/1, Delay477/1
  Relational173/1 -> Delay390/1
  AddSub131/1 -> Mux129/3
  Delay526/1 -> Relational173/1, Delay530/1
  Delay247/1 -> Mux141/1
  Delay341/1 -> Delay401/1, Relational182/1
  Mux166/1 -> AddSub169/1, Delay516/1
  Relational141/1 -> Delay251/1
  Relational116/1 -> Delay593/1
  logi_b68/1 -> Relational144/2, Relational143/2
  Mux140/1 -> Delay333/1, AddSub145/1
  Delay380/1 -> Mux146/2
  logi_b74/1 -> Relational150/2, Relational158/2
  Delay375/1 -> Mux145/1
  AddSub189/1 -> Mux188/3
  Mux174/1 -> AddSub177/1, Delay474/1
  Delay337/1 -> Mux96/2
  AddSub121/1 -> Mux119/3
  Delay489/1 -> Relational184/1, Delay492/1
  AddSub163/1 -> Mux170/3
  Mux144/1 -> AddSub148/1, Delay376/1
  Delay586/1 -> Mux114/2
  Delay397/1 -> Mux160/1
  Delay542/1 -> Mux124/2
  Mux126/1 -> AddSub183/1, Delay245/1
  Delay529/1 -> Mux181/2
  Delay525/1 -> Mux169/2
  Delay550/1 -> Mux127/2
  Delay354/1 -> Mux152/2
  Delay248/1 -> Mux141/2
  Relational154/1 -> Delay350/1
  Relational199/1 -> Delay442/1
  AddSub181/1 -> Mux178/3
  Delay458/1 -> Mux102/1
  Mux95/1 -> AddSub99/1, Delay209/1
  Delay377/1 -> Delay378/1, Relational148/1
  Delay388/1 -> Relational160/1, Delay344/1
  AddSub124/1 -> Mux122/3
  Relational189/1 -> Delay504/1
  logi_b69/1 -> Relational145/2, Relational151/2
  Delay362/1 -> Mux154/2
  Delay378/1 -> Delay381/1, Relational149/1
  Delay473/1 -> Mux183/1
  AddSub188/1 -> Mux187/3
  Delay423/1 -> Mux163/2
  AddSub98/1 -> Mux95/3
  Mux162/1 -> AddSub165/1, Delay491/1
  Mux173/1 -> AddSub176/1, Delay469/1
  logi_b75/1 -> Relational153/2, Relational159/2
  Delay428/1 -> Relational101/1, Delay432/1
  Relational150/1 -> Delay386/1
  Delay480/1 -> Mux177/2
  Delay585/1 -> Mux114/1
  logi_b78/1 -> Relational177/2, Relational192/2
  Delay570/1 -> Delay573/1, Relational136/1
  Mux182/1 -> AddSub192/1, Delay411/1
  AddSub195/1 -> Mux163/3
  Relational115/1 -> Delay590/1
  Relational137/1 -> Delay578/1
  Relational185/1 -> Delay446/1
  Delay517/1 -> Mux120/2
  logi_b71/1 -> Relational147/2, Relational155/2
  Delay590/1 -> Mux115/1
  Delay210/1 -> Mux130/1
  Mux153/1 -> AddSub156/1, Delay362/1
  Delay415/1 -> Delay436/1, Relational197/1
  Delay511/1 -> Relational167/1, Delay514/1
  Delay484/1 -> Mux183/2
  Delay492/1 -> Relational186/1, Delay496/1
  Relational171/1 -> Delay527/1
  Delay557/1 -> Mux95/1
  AddSub106/1 -> Mux102/3
  Delay358/1 -> Mux153/2
  Delay589/1 -> Delay592/1, Relational116/1
  Relational174/1 -> Delay429/1
  Delay350/1 -> Mux151/1
  AddSub200/1 -> Mux197/3
  Delay420/1 -> Delay424/1, Relational200/1
  logi_b76/1 -> Relational160/2, Relational161/2
  Relational151/1 -> Delay340/1
  logi_b70/1 -> Relational146/2, Relational154/2
  AddSub107/1 -> Mux103/3
  logi_b67/1 -> Relational140/2, Relational142/2
  Delay367/1 -> Mux156/1
  Mux168/1 -> AddSub171/1, Delay525/1
  AddSub154/1 -> Mux149/3
  Relational146/1 -> Delay372/1
  Delay442/1 -> Mux197/1
  Mux133/1 -> AddSub135/1, Delay572/1
  Delay414/1 -> Mux193/2
  Mux170/1 -> AddSub173/1, Delay419/1
  Relational147/1 -> Delay375/1
  Mux104/1 -> AddSub101/1, Delay558/1
  AddSub180/1 -> Mux190/3
  Mux192/1 -> Delay418/1, AddSub104/1
  Mux113/1 -> AddSub117/1, Delay586/1
  AddSub134/1 -> Mux133/3
  Delay583/1 -> Mux113/2
  Delay569/1 -> Mux133/2
  AddSub118/1 -> Mux115/3
  Relational176/1 -> Delay487/1
  Delay559/1 -> Relational132/1, Delay562/1
  Mux131/1 -> AddSub132/1, Delay564/1
  Delay457/1 -> Relational175/1, Delay460/1
  Relational112/1 -> Delay224/1
  Delay436/1 -> Relational198/1, Delay441/1
  Delay394/1 -> Mux164/2
  Relational133/1 -> Delay563/1
  Delay591/1 -> Mux115/2
  Delay500/1 -> Delay503/1, Relational189/1
  Delay496/1 -> Delay497/1, Relational187/1
  Delay587/1 -> Delay589/1, Relational115/1
  AddSub136/1 -> Mux135/3
  logi_b92/1 -> Relational173/2, Relational190/2
  Delay515/1 -> Mux167/1
  Delay459/1 -> Mux102/2
  Relational162/1 -> Delay402/1
  Relational144/1 -> Delay332/1
  Mux187/1 -> AddSub189/1, Delay505/1
  Delay488/1 -> Mux162/2
  Delay223/1 -> Delay581/1, Relational112/1
  Relational113/1 -> Delay582/1
  AddSub123/1 -> Mux121/3
  Delay467/1 -> Relational178/1, Delay470/1
  Mux156/1 -> AddSub160/1, Delay343/1
  Delay222/1 -> Delay547/1, Relational37/1
  Delay553/1 -> Mux119/1
  Delay594/1 -> Mux116/2
  Delay439/1 -> Relational196/1, Delay462/1
  Relational193/1 -> Delay406/1
  AddSub116/1 -> Mux113/3
  Delay592/1 -> Delay595/1, Relational117/1
  Relational121/1 -> Delay553/1
  Relational130/1 -> Delay588/1
  Relational136/1 -> Delay574/1
  Delay462/1 -> Relational122/1, Delay495/1
  Mux197/1 -> AddSub138/1, Delay234/1
  Mux184/1 -> AddSub185/1, Delay494/1
  Mux130/1 -> AddSub141/1, Delay253/1
  Mux146/1 -> AddSub151/1, Delay384/1
  Mux191/1 -> Delay414/1, AddSub197/1
  Delay573/1 -> Relational137/1, Delay576/1
  Delay519/1 -> Mux170/1
  Delay334/1 -> Delay370/1, Relational145/1
  Relational145/1 -> Delay335/1
  AddSub133/1 -> Mux130/3
  Delay544/1 -> Mux125/1
  AddSub127/1 -> Mux125/3
  logi_b80/1 -> Relational179/2, Relational102/2
  Delay478/1 -> Relational183/1, Delay481/1
  logi_b51/1 -> Relational130/2, Relational124/2
  Delay497/1 -> Delay500/1, Relational188/1
  AddSub139/1 -> Mux150/3
  Relational129/1 -> Delay544/1
  AddSub140/1 -> Mux138/3
  Mux132/1 -> AddSub134/1, Delay569/1
  Mux135/1 -> AddSub137/1, Delay579/1
  AddSub165/1 -> Mux184/3
  Mux112/1 -> AddSub116/1, Delay583/1
  Mux127/1 -> Delay226/1, AddSub194/1
  logi_b86/1 -> Relational166/2, Relational172/2
  Delay402/1 -> Mux103/1
  Relational172/1 -> Delay400/1
  Delay386/1 -> Mux148/1
  Relational106/1 -> Delay458/1
  Delay363/1 -> Relational159/1, Delay366/1
  Mux151/1 -> AddSub153/1, Delay354/1
  AddSub147/1 -> Mux144/3
  Delay477/1 -> Mux176/2
  AddSub144/1 -> Mux151/3
  Relational138/1 -> Delay231/1
  AddSub172/1 -> Mux183/3
  Delay430/1 -> Mux200/1
  Delay422/1 -> Delay439/1, Relational185/1
  AddSub149/1 -> Mux146/3
  Constant2/1 -> AddSub31/2, AddSub9/2, AddSub11/2, AddSub33/2, AddSub35/2, AddSub36/2, AddSub37/2, AddSub60/2, AddSub44/2, AddSub52/2, AddSub54/2, AddSub55/2, AddSub56/2, AddSub59/2, AddSub79/2, AddSub112/2, AddSub63/2, AddSub81/2, AddSub83/2, AddSub84/2, AddSub85/2, AddSub109/2, AddSub130/2, AddSub194/2, AddSub105/2, AddSub132/2, AddSub134/2, AddSub135/2, AddSub136/2, AddSub162/2, AddSub144/2, AddSub153/2, AddSub155/2, AddSub156/2, AddSub157/2, AddSub160/2, AddSub182/2, AddSub113/2, AddSub165/2, AddSub185/2, AddSub187/2, AddSub188/2, AddSub189/2, AddSub104/2, AddSub196/2, AddSub238/2, AddSub205/2, AddSub294/2, AddSub293/2, AddSub207/2, AddSub291/2, AddSub288/2, AddSub287/2, AddSub286/2, AddSub285/2, AddSub283/2, AddSub263/2, AddSub262/2, AddSub211/2, AddSub280/2, AddSub209/2, AddSub206/2, AddSub299/2, AddSub289/2, AddSub278/2, AddSub271/2, AddSub261/2, AddSub258/2, AddSub256/2, AddSub255/2, AddSub254/2, AddSub140/2, AddSub102/2, AddSub195/2, AddSub193/2, AddSub190/2, AddSub164/2, AddSub106/2, AddSub103/2, AddSub201/2, AddSub191/2, AddSub180/2, AddSub173/2, AddSub163/2, AddSub158/2, AddSub143/2, AddSub142/2, AddSub137/2, AddSub101/2, AddSub172/2, AddSub161/2, AddSub150/2, AddSub139/2, AddSub128/2, AddSub120/2, AddSub99/2, AddSub98/2, AddSub40/2, AddSub100/2, AddSub91/2, AddSub90/2, AddSub89/2, AddSub86/2, AddSub62/2, AddSub110/2, AddSub108/2, AddSub97/2, AddSub87/2, AddSub77/2, AddSub70/2, AddSub61/2, AddSub57/2, AddSub43/2, AddSub42/2, AddSub38/2, AddSub10/2, AddSub7/2, AddSub6/2, AddSub5/2, AddSub4/2, AddSub3/2, AddSub2/2, AddSub1/2, AddSub/2, Mux/3
  Delay522/1 -> Mux168/2
  Delay441/1 -> Relational199/1, Delay444/1
  Delay333/1 -> Mux142/2
  Delay244/1 -> Relational38/1, Delay552/1
  AddSub299/1 -> Mux204/3
  logi_b110/1 -> Relational262/2, Relational275/2
  logi_b109/1 -> Relational283/2, Relational210/2
  Delay726/1 -> Relational238/1
  Relational259/1 -> Delay661/1
  Delay747/1 -> Mux204/2
  Relational264/1 -> Delay691/1
  AddSub291/1 -> Mux292/3
  Delay734/1 -> Mux296/2
  Delay760/1 -> Mux273/2
  AddSub205/1 -> Mux300/3
  Delay624/1 -> Mux249/1
  Delay758/1 -> Relational277/1, Delay761/1
  AddSub250/1 -> Mux248/3
  Relational206/1 -> Delay742/1
  Delay613/1 -> Mux237/1
  Delay718/1 -> Relational302/1, Delay722/1
  Mux281/1 -> AddSub284/1, Delay685/1
  AddSub288/1 -> Mux289/3
  Relational283/1 -> Delay776/1
  logi_b120/1 -> Relational295/2, Relational294/2
  logi_b121/1 -> Relational297/2, Relational300/2
  Delay662/1 -> Mux256/2
  Relational292/1 -> Delay703/1
  Delay763/1 -> Mux274/2
  AddSub267/1 -> Mux267/3
  Delay658/1 -> Mux255/1
  Delay432/1 -> Relational138/1, Delay610/1
  Delay715/1 -> Mux263/1
  Delay705/1 -> Mux291/2
  Relational290/1 -> Delay802/1
  Delay785/1 -> Mux284/2
  logi_b115/1 -> Relational269/2, Relational287/2
  Mux286/1 -> AddSub286/1, Delay796/1
  Delay787/1 -> Mux285/1
  Delay814/1 -> Delay817/1, Relational270/1
  AddSub249/1 -> Mux247/3
  Delay737/1 -> Mux297/2
  AddSub282/1 -> Mux281/3
  Delay721/1 -> Mux299/2
  Delay625/1 -> Mux249/2
  logi_b105/1 -> Relational278/2, Relational301/2
  Delay788/1 -> Mux285/2
  AddSub262/1 -> Mux262/3
  AddSub269/1 -> Mux269/3
  AddSub264/1 -> Mux264/3
  Mux263/1 -> AddSub294/1, Delay721/1
  Relational203/1 -> Delay655/1
  Delay700/1 -> Mux292/1
  Mux258/1 -> Delay683/1, AddSub261/1
  Delay704/1 -> Mux291/1
  Mux204/1 -> AddSub206/1, Delay750/1
  Delay765/1 -> Delay769/1, Relational280/1
  Relational287/1 -> Delay792/1
  Delay701/1 -> Mux292/2
  Mux271/1 -> AddSub273/1, Delay760/1
  Mux277/1 -> AddSub279/1, Delay777/1
  Relational301/1 -> Delay727/1
  logi_b111/1 -> Relational265/2, Relational264/2
  Delay697/1 -> Mux207/2
  Delay711/1 -> Mux259/1
  Relational288/1 -> Delay795/1
  Delay817/1 -> Delay820/1, Relational271/1
  Delay659/1 -> Mux255/2
  Delay739/1 -> Delay741/1, Relational206/1
  Delay803/1 -> Mux289/2
  Relational295/1 -> Delay706/1
  Delay712/1 -> Mux259/2
  AddSub297/1 -> Mux296/3
  Mux254/1 -> AddSub255/1, Delay659/1
  Delay614/1 -> Mux237/2
  Relational253/1 -> Delay624/1
  AddSub256/1 -> Mux256/3
  Delay764/1 -> Delay765/1, Relational279/1
  Delay713/1 -> Mux280/2
  Delay780/1 -> Relational265/1, Delay689/1
  Delay660/1 -> Relational261/1, Delay635/1
  Mux260/1 -> AddSub262/1, Delay782/1
  Mux290/1 -> AddSub289/1, Delay743/1
  Relational286/1 -> Delay787/1
  AddSub283/1 -> Mux285/3
  Mux300/1 -> AddSub238/1, Delay612/1
  Delay679/1 -> Relational253/1, Delay682/1
  AddSub285/1 -> Mux286/3
  Delay807/1 -> Mux266/2
  Delay798/1 -> Mux288/1
  Delay684/1 -> Mux282/1
  Relational302/1 -> Delay720/1
  Delay762/1 -> Mux274/1
  Relational268/1 -> Delay809/1
  Delay703/1 -> Mux280/1
  AddSub272/1 -> Mux271/3
  Delay812/1 -> Delay814/1, Relational269/1
  Mux205/1 -> AddSub209/1, Delay753/1
  Delay821/1 -> Mux281/1
  AddSub254/1 -> Mux254/3
  Mux206/1 -> AddSub280/1, Delay779/1
  Relational277/1 -> Delay759/1
  Relational284/1 -> Delay784/1
  AddSub277/1 -> Mux277/3
  Delay775/1 -> Relational262/1, Delay780/1
  Delay444/1 -> Relational139/1, Delay617/1
  AddSub289/1 -> Mux298/3
  Mux259/1 -> AddSub293/1, Delay717/1
  Mux249/1 -> AddSub257/1, Delay640/1
  Delay799/1 -> Mux288/2
  logi_b119/1 -> Relational291/2, Relational293/2
  Relational278/1 -> Delay762/1
  Delay742/1 -> Mux298/1
  AddSub294/1 -> Mux299/3
  Relational208/1 -> Delay749/1
  Relational291/1 -> Delay704/1
  Delay640/1 -> Mux257/2
  Relational275/1 -> Delay755/1
  Delay719/1 -> Relational301/1, Delay739/1
  Mux257/1 -> Delay757/1, AddSub272/1
  Delay749/1 -> Mux205/1
  AddSub273/1 -> Mux273/3
  Delay741/1 -> Delay744/1, Relational207/1
  Delay796/1 -> Mux287/2
  logi_b103/1 -> Relational276/2, Relational282/2
  AddSub211/1 -> Mux260/3
  logi_b113/1 -> Relational267/2, Relational284/2
  Delay804/1 -> Mux265/2
  AddSub284/1 -> Mux282/3
  Delay776/1 -> Mux278/1
  Delay797/1 -> Relational290/1, Delay801/1
  Relational204/1 -> Delay677/1
  Delay681/1 -> Mux248/2
  AddSub274/1 -> Mux274/3
  AddSub268/1 -> Mux268/3
  Delay766/1 -> Mux275/1
  Relational260/1 -> Delay639/1
  AddSub257/1 -> Mux257/3
  AddSub275/1 -> Mux275/3
  Relational298/1 -> Delay732/1
  Delay781/1 -> Mux271/1
  Delay770/1 -> Mux276/1
  Delay746/1 -> Mux204/1
  Delay738/1 -> Relational239/1
  Relational300/1 -> Delay715/1
  Delay743/1 -> Mux298/2
  Relational266/1 -> Delay690/1
  Delay748/1 -> Relational210/1, Delay751/1
  Delay677/1 -> Mux247/1
  Mux276/1 -> AddSub277/1, Delay774/1
  Mux269/1 -> AddSub282/1, Delay823/1
  Delay801/1 -> Relational293/1, Delay699/1
  Relational297/1 -> Delay710/1
  Mux248/1 -> AddSub252/1, Delay625/1
  Delay754/1 -> Relational264/1, Delay693/1
  Relational265/1 -> Delay686/1
  Delay769/1 -> Delay772/1, Relational281/1
  Delay777/1 -> Mux278/2
  Delay612/1 -> Mux238/2
  Mux207/1 -> Delay688/1, AddSub264/1
  Mux289/1 -> AddSub291/1, Delay701/1
  Delay824/1 -> Relational291/1, Delay702/1
  logi_b117/1 -> Relational271/2, Relational289/2
  Mux293/1 -> AddSub296/1, Delay729/1
  logi_b108/1 -> Relational281/2, Relational208/2
  Mux280/1 -> AddSub278/1, Delay731/1
  Mux285/1 -> AddSub285/1, Delay793/1
  Delay639/1 -> Mux257/1
  AddSub265/1 -> Mux265/3
  logi_b116/1 -> Relational270/2, Relational288/2
  Mux288/1 -> AddSub288/1, Delay803/1
  AddSub276/1 -> Mux276/3
  Delay802/1 -> Mux289/1
  Delay720/1 -> Mux299/1
  Delay706/1 -> Mux293/1
  Relational207/1 -> Delay746/1
  Delay725/1 -> Mux300/2
  Delay686/1 -> Mux264/1
  Mux295/1 -> AddSub297/1, Delay734/1
  Delay699/1 -> Relational294/1, Delay714/1
  Delay727/1 -> Mux290/1
  Delay795/1 -> Mux287/1
  Relational239/1 -> Delay613/1
  Mux267/1 -> AddSub268/1, Delay816/1
  Delay759/1 -> Mux273/1
  Delay611/1 -> Mux238/1
  Delay773/1 -> Mux277/1
  AddSub236/1 -> Mux237/3
  AddSub255/1 -> Mux255/3
  Delay744/1 -> Delay748/1, Relational208/1
  Delay779/1 -> Mux279/2
  Mux298/1 -> AddSub299/1, Delay747/1
  logi_b124/1 -> Relational239/2, Relational238/2
  Relational280/1 -> Delay770/1
  Delay638/1 -> Delay758/1, Relational276/1
  Delay694/1 -> Mux262/1
  Delay689/1 -> Delay805/1, Relational266/1
  Delay808/1 -> Relational268/1, Delay812/1
  Mux296/1 -> AddSub298/1, Delay737/1
  Mux255/1 -> AddSub256/1, Delay662/1
  AddSub206/1 -> Mux205/3
  Delay693/1 -> Delay783/1, Relational272/1
  Delay695/1 -> Relational292/1, Delay719/1
  Delay793/1 -> Mux286/2
  Delay768/1 -> Mux275/2
  Relational282/1 -> Delay813/1
  Delay755/1 -> Mux279/1
  Delay792/1 -> Mux286/1
  Delay683/1 -> Mux270/2
  Delay655/1 -> Mux254/1
  Mux279/1 -> Delay692/1, AddSub211/1
  Delay710/1 -> Mux295/1
  Delay757/1 -> Mux271/2
  Delay637/1 -> Mux258/2
  Mux247/1 -> AddSub250/1, Delay681/1
  Delay784/1 -> Mux284/1
  Delay690/1 -> Mux265/1
  Mux265/1 -> AddSub266/1, Delay807/1
  AddSub266/1 -> Mux266/3
  Mux299/1 -> AddSub205/1, Delay725/1
  AddSub296/1 -> Mux295/3
  Delay815/1 -> Mux268/1
  logi_b123/1 -> Relational299/2, Relational205/2
  Relational258/1 -> Delay658/1
  Relational267/1 -> Delay806/1
  Relational279/1 -> Delay766/1
  AddSub290/1 -> Mux291/3
  Delay729/1 -> Mux295/2
  Delay731/1 -> Mux290/2
  Delay806/1 -> Mux266/1
  Delay692/1 -> Mux260/2
  logi_b122/1 -> Relational298/2, Relational302/2
  Mux278/1 -> AddSub210/1, Delay697/1
  AddSub280/1 -> Mux279/3
  Delay636/1 -> Mux258/1
  Relational270/1 -> Delay818/1
  Relational281/1 -> Delay773/1
  Relational269/1 -> Delay815/1
  AddSub271/1 -> Mux280/3
  AddSub258/1 -> Mux258/3
  Mux264/1 -> AddSub265/1, Delay804/1
  AddSub295/1 -> Mux293/3
  Relational294/1 -> Delay711/1
  Delay818/1 -> Mux269/1
  Delay702/1 -> Relational295/1, Delay709/1
  Delay810/1 -> Mux267/2
  logi_b107/1 -> Relational280/2, Relational207/2
  AddSub207/1 -> Mux259/3
  Delay685/1 -> Mux282/2
  Relational205/1 -> Delay724/1
  Delay750/1 -> Mux205/2
  logi_b114/1 -> Relational268/2, Relational286/2
  Delay732/1 -> Mux296/1
  Delay678/1 -> Mux247/2
  Relational261/1 -> Delay636/1
  Mux275/1 -> AddSub276/1, Delay771/1
  Relational273/1 -> Delay684/1
  Delay820/1 -> Relational273/1, Delay824/1
  Delay635/1 -> Delay695/1, Relational282/1
  Mux266/1 -> AddSub267/1, Delay810/1
  logi_b100/1 -> Relational250/2, Relational258/2
  AddSub287/1 -> Mux288/3
  Mux274/1 -> AddSub275/1, Delay768/1
  Delay783/1 -> Relational284/1, Delay786/1
  AddSub261/1 -> Mux270/3
  Delay691/1 -> Mux260/1
  Delay823/1 -> Mux281/2
  Delay819/1 -> Mux269/2
  Relational299/1 -> Delay736/1
  AddSub279/1 -> Mux278/3
  Delay752/1 -> Mux206/1
  Delay682/1 -> Relational260/1, Delay638/1
  Relational289/1 -> Delay798/1
  Delay656/1 -> Mux254/2
  AddSub286/1 -> Mux287/3
  Delay717/1 -> Mux263/2
  Mux262/1 -> AddSub263/1, Delay785/1
  Mux273/1 -> AddSub274/1, Delay763/1
  logi_b101/1 -> Relational253/2, Relational259/2
  Delay722/1 -> Relational205/1, Delay726/1
  Relational250/1 -> Delay680/1
  Delay774/1 -> Mux277/2
  logi_b104/1 -> Relational277/2, Relational292/2
  Mux282/1 -> AddSub290/1, Delay705/1
  AddSub293/1 -> Mux263/3
  Delay709/1 -> Delay730/1, Relational297/1
  Delay805/1 -> Relational267/1, Delay808/1
  Delay786/1 -> Relational286/1, Delay790/1
  Relational271/1 -> Delay821/1
  AddSub209/1 -> Mux206/3
  AddSub298/1 -> Mux297/3
  Delay714/1 -> Delay718/1, Relational300/1
  logi_b102/1 -> Relational260/2, Relational261/2
  AddSub210/1 -> Mux207/3
  Delay661/1 -> Mux256/1
  Mux268/1 -> AddSub269/1, Delay819/1
  AddSub252/1 -> Mux249/3
  Delay736/1 -> Mux297/1
  Delay708/1 -> Mux293/2
  Mux270/1 -> AddSub271/1, Delay713/1
  AddSub278/1 -> Mux290/3
  Mux292/1 -> Delay712/1, AddSub207/1
  Relational276/1 -> Delay781/1
  Delay751/1 -> Relational275/1, Delay754/1
  Delay730/1 -> Relational298/1, Delay735/1
  Delay688/1 -> Mux264/2
  Delay794/1 -> Delay797/1, Relational289/1
  Delay790/1 -> Delay791/1, Relational287/1
  logi_b118/1 -> Relational273/2, Relational290/2
  Delay809/1 -> Mux267/1
  Delay753/1 -> Mux206/2
  Relational262/1 -> Delay696/1
  Mux287/1 -> AddSub287/1, Delay799/1
  Delay782/1 -> Mux262/2
  Delay761/1 -> Relational278/1, Delay764/1
  Mux256/1 -> AddSub258/1, Delay637/1
  Relational293/1 -> Delay700/1
  Mux297/1 -> AddSub236/1, Delay614/1
  Mux284/1 -> AddSub283/1, Delay788/1
  Mux291/1 -> Delay708/1, AddSub295/1
  Delay813/1 -> Mux270/1
  logi_b106/1 -> Relational279/2, Relational206/2
  Delay772/1 -> Relational283/1, Delay775/1
  Delay791/1 -> Delay794/1, Relational288/1
  AddSub238/1 -> Mux238/3
  AddSub263/1 -> Mux284/3
  logi_b112/1 -> Relational266/2, Relational272/2
  Delay696/1 -> Mux207/1
  Relational272/1 -> Delay694/1
  Delay680/1 -> Mux248/1
  Relational210/1 -> Delay752/1
  Delay657/1 -> Relational259/1, Delay660/1
  Delay771/1 -> Mux276/2
  Relational238/1 -> Delay611/1
  Delay724/1 -> Mux300/1
  Delay816/1 -> Mux268/2
  Delay735/1 -> Relational299/1, Delay738/1
  Mux237/1 -> Slice1/1
  Mux138/1 -> AddSub254/1, Delay656/1
  logi_b99/1 -> Relational204/2, Relational203/2
  Mux137/1 -> AddSub249/1, Delay678/1
  Delay547/1 -> Relational95/1, Delay577/1
  Mux238/1 -> Slice/1
  Gateway Out/1 -> Output/1
  Constant5/1 -> Delay604/1
  Delay604/1 -> AddSub22/2
  Slice/1 -> Delay60/1, AddSub18/1, Delay59/1
  Delay610/1 -> Relational203/1, Delay615/1
  Delay615/1 -> Relational258/1, Delay657/1
  Delay616/1 -> Relational250/1, Delay679/1
  Delay617/1 -> Relational204/1, Delay616/1
  ROM2/1 -> Concat/2
  ROM3/1 -> Concat/3
  ROM4/1 -> Concat/4
  ROM1/1 -> Concat/1
  ROM7/1 -> Concat/7
  Concat/1 -> Scaling/1
  ROM5/1 -> Concat/5
  ROM6/1 -> Concat/6
  ROM8/1 -> Concat/8
  ROM10/1 -> Concat/10
  ROM11/1 -> Concat/11
  ROM9/1 -> Concat/9
  ROM14/1 -> Concat/14
  ROM13/1 -> Concat/13
  ROM15/1 -> Concat/15
  ROM12/1 -> Concat/12
  ROM16/1 -> Concat/16
  ROM22/1 -> Concat/22
  ROM32/1 -> Concat/32
  ROM31/1 -> Concat/31
  ROM26/1 -> Concat/26
  ROM30/1 -> Concat/30
  Slice3/1 -> ROM31/1, ROM32/1, ROM30/1, ROM29/1, ROM28/1, ROM27/1, ROM26/1, ROM25/1, ROM24/1, ROM23/1, ROM22/1, ROM21/1, ROM20/1, ROM19/1, ROM18/1, ROM17/1, ROM16/1, ROM15/1, ROM14/1, ROM13/1, ROM12/1, ROM11/1, ROM10/1, ROM9/1, ROM4/1, ROM1/1, ROM2/1, ROM3/1, ROM5/1, ROM6/1, ROM7/1, ROM8/1
  ROM29/1 -> Concat/29
  ROM27/1 -> Concat/27
  ROM21/1 -> Concat/21
  ROM20/1 -> Concat/20
  ROM23/1 -> Concat/23
  ROM25/1 -> Concat/25
  ROM17/1 -> Concat/17
  ROM28/1 -> Concat/28
  ROM19/1 -> Concat/19
  ROM18/1 -> Concat/18
  ROM24/1 -> Concat/24
  Slice1/1 -> Delay61/1
